simulink model "W01_Base_Map_cs"  (R2019a)
settings: Solver=FixedStepDiscrete  StartTime=0.0  StopTime=inf  FixedStep=1/20  RelTol=1e-3
PreLoadFcn:
  | mbxruntime.callbacks.PreLoadFcn(bdroot);
  | check_NUTS_defined
  | model_closed = 0;
  | assignin('base',['model_closed_' bdroot],false);
PostLoadFcn:
  | mbxruntime.callbacks.PostLoadFcn(bdroot);
InitFcn:
  | mbxruntime.callbacks.InitFcn(bdroot);
StartFcn:
  | mbxruntime.callbacks.StartFcn(bdroot);
StopFcn:
  | mbxruntime.callbacks.StopFcn(bdroot);;
  | 
model workspace: external: MAT-File (data not in the file)
undefined symbols (not defined in the file or in its folder): actors_poses, adeye_msgs, categorized_poses, DiscIntNeverNeededParam, geometry_msgs, Header, InitImageOutputDir, mbxruntime, pose_otherCar, PoseArray, Poses, Poses_SL_Info, tabledata, W01_Base_Map_cs_004987d4dd39f9b6, W01_Base_Map_cs_00cc66853e964a64, W01_Base_Map_cs_00f75b713170549a, W01_Base_Map_cs_01472650a6655f66, W01_Base_Map_cs_021eada97d6d5412, W01_Base_Map_cs_0288936122941f67, W01_Base_Map_cs_03728bc5c0f611d1, W01_Base_Map_cs_03729b7883682eca, W01_Base_Map_cs_03935175e827b825, W01_Base_Map_cs_03ecb5a7ceaf36f1, W01_Base_Map_cs_04544dd62153117c, W01_Base_Map_cs_04f0838a8dce3a91, W01_Base_Map_cs_05c6883b663017e6, W01_Base_Map_cs_074ff6b44c8e4b42, W01_Base_Map_cs_0850adb5f9b52847, W01_Base_Map_cs_09b4416d284a38c0, W01_Base_Map_cs_09f1a8cccf5dc476, W01_Base_Map_cs_0a863e6a78242047, W01_Base_Map_cs_0b51b2edfb6b21eb, W01_Base_Map_cs_0c25b2d8edd3fbea, W01_Base_Map_cs_0cec291d859792a3, W01_Base_Map_cs_0d48999ceb9def0a, W01_Base_Map_cs_1054e386bc2b89f8, W01_Base_Map_cs_129d7fd29679c9e4, W01_Base_Map_cs_1557dafebe6eb5e3, W01_Base_Map_cs_155bf6da17508b9f, W01_Base_Map_cs_1619aae3285d69a6, W01_Base_Map_cs_18faf784f59d6ded, W01_Base_Map_cs_190ae931cd3b3df1, W01_Base_Map_cs_1a47612a95ab18a1, W01_Base_Map_cs_1a96581334d27a16, W01_Base_Map_cs_1b9c28e1ad91b987, W01_Base_Map_cs_1bd80946b29cc249, W01_Base_Map_cs_1bf8c5472ecd97cc, W01_Base_Map_cs_1c047b8f6e9a46e9, W01_Base_Map_cs_1c4e91c4c8848966, W01_Base_Map_cs_1dfe629d3c3a34d6, W01_Base_Map_cs_1e00e80d4fa95f87, W01_Base_Map_cs_1e67a7d0e7e33a10, W01_Base_Map_cs_1e994bb86296e53e, W01_Base_Map_cs_1f3d28b65a209a81, W01_Base_Map_cs_1f4ddfcaed2bdfa2, W01_Base_Map_cs_20e6a062a8bf989a, W01_Base_Map_cs_210ba2feda70a68e, W01_Base_Map_cs_211f71a4af886b52, W01_Base_Map_cs_2177d1459a678375, W01_Base_Map_cs_21a90c8036f5a434 ... (+289)
libraries: PreScanSimulinkLibrary x112, robotcorelib x55, adeye_lib x46, simulink x31, simulink_extras x24, robotlib x3, PreScanUsefulBlocks x1
(part 1 of 32)
CloseFcn:
  | mbxruntime.callbacks.CloseFcn(bdroot);
  | evalin('base',['clear model_closed_' bdroot]);
  | model_closed = 1;
settings Model: Creator=PRESCAN  LastModifiedBy=adeye
settings DataIOCC: LimitDataPoints=on  SaveFormat=Array  SignalLoggingSaveFormat=ModelDataLogs  ReturnWorkspaceOutputs=off
settings OptimizationCC: DefaultParameterBehavior=Inlined  ExpressionDepthLimit=2147483647  InitFltsAndDblsToZero=on  LifeSpan=inf
settings DebuggingCC: SaveWithParameterizedLinksMsg=none  UnderspecifiedInitializationDetection=Classic  MergeDetectMultiDrivingBlocksExec=none  SignalResolutionControl=TryResolveAllWithWarning  MultiTaskDSMMsg=warning  MultiTaskCondExecSysMsg=none  FcnCallInpInsideContextMsg=warning  StateNameClashWarn=warning  SFUnexpectedBacktrackingDiag=warning  SFNoUnconditionalDefaultTransitionDiag=warning  SFExecutionAtInitializationDiag=none  ArithmeticOperatorsInVariantConditions=warning
settings HardwareCC: ProdBitPerPointer=32  ProdBitPerSizeT=32  ProdBitPerPtrDiffT=32  ProdLargestAtomicFloat=None  ProdIntDivRoundTo=Undefined  ProdEndianess=Unspecified  ProdWordSize=32  ProdHWDeviceType=32-bit Generic
settings ModelReferenceCC: UpdateModelReferenceTargets=IfOutOfDate  PropagateSignalLabelsOutOfModel=off
settings SFSimCC: SimUseLocalCustomCode=off  SimParseCustomCode=off
settings SFSimCC: SimCustomHeaderCode=|
  | #include "prescan.h"
  | #include "prescan_platform.h"
  | #include "prescan_aimsunturnindicatorsetter_data.h"
settings RTWCC: RTWUseLocalCustomCode=off
settings CodeAppCC: StateflowObjectComments=on
settings GRTTargetCC: TargetFcnLib=ansi_tfl_tmw.mat  TargetLangStandard=C89/C90 (ANSI)  GeneratePreprocessorConditionals=Disable all  CombineOutputUpdateFcns=off  GRTInterface=on
settings ConfigComp: CovMetricSettings=dw  CovHtmlReporting=on  CovSaveCumulativeToWorkspaceVar=on  CovSaveSingleToWorkspaceVar=on  CovExternalEMLEnable=off  CovSFcnEnable=off

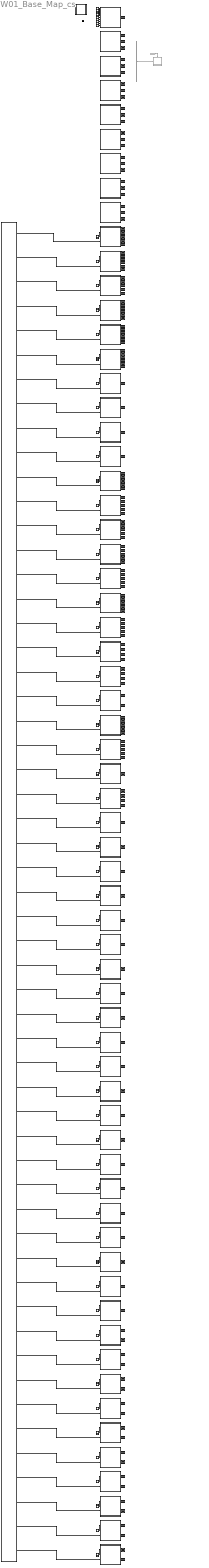
== system W01_Base_Map_cs ==
  note: Regenerate
  note: Simulink Mode
  note: Open Useful Blocks
  note: 2020.4.0
  note: Version:
  note: Author(s):
  note: Adeye
  note: Descriptive text:
  note: N.A.
  note: Demo Help
  note: ====== Num ID ====== 91 93 94 95 96 97 76 77 78 79 80 82 83 81 37 109 115 116 117 118 119 120 121 122 123 124 125 126 127 128 ====== Num ID ====== 129 130 131 132 133 134 135 136 137 138 139 140 141 142 143 144 145 146 147 148 149 150 151 152 153 154 155 156 157 110 ====== Num ID ====== 159 160 161 162 163 164 165 166 167
  note: ============= OBU-Beacon ID ============= ============= OBU-Beacon ID ============= ============= OBU-Beacon ID =============
  note: ======= Type ID ======= 12 12 12 12 12 12 15 15 15 15 15 15 15 15 4 4 4 4 4 4 2 2 1 1 4 4 4 4 4 4 ======= Type ID ======= 4 4 4 4 4 4 4 4 1 1 1 1 1 1 1 1 1 1 1 1 1 1 1 1 1 1 2 2 2 4 ======= Type ID ======= 4 4 4 4 4 4 4 4 4
  note: ================ Type Tag ================ Building Building Building Building Building Building Animated traffic sign Animated traffic sign Animated traffic sign Animated traffic sign Animated traffic sign Animated traffic sign Animated traffic sign Animated traffic sign Human Human Human Human Human Human Motor Motor Car Car Human Human Human Human Human Human ================ Type Tag ================ Human Human Human Human Human Human Human Human Car Car Car Car Car Car Car Car Car Car Car Car Car Car Car Car Car Car Motor Motor Motor Human ================ Type Tag ================ Human Human Human Human Human Human Human Human Human
  note: == SD == Y Y Y Y Y Y Y Y Y Y Y Y Y Y Y Y Y Y Y Y Y Y Y Y Y Y Y Y Y Y == SD == Y Y Y Y Y Y Y Y Y Y Y Y Y Y Y Y Y Y Y Y Y Y Y Y Y Y Y Y Y Y == SD == Y Y Y Y Y Y Y Y Y
  note: == CD == N N N N N N N N N N N N N N N N N N N N N N N N N N N N N N == CD == N N N N N N N N N N N N N N N N N N N N N N N N N N N N N N == CD == N N N N N N N N N
  note: ================================== Name ================================== HouseOld3_1 HouseOld4_1 HouseOld5_1 School_1 OfficeBrownFlat_1 OfficeBrownTall2_1 TrafficLightRoadSideNL_1 TrafficLightRoadSideNL_2 TrafficLightRoadSideNL_3 TrafficLightRoadSideNL_4 TrafficLightRoadSideNL_5 TrafficLightRoadSideNL_7 TrafficLightRoadSideNL_8 TrafficLightRoadSideNL_6 Female_Regular_1 Male_wLargeBackpack_1 Male_wBackpack_1 Male_ShoppingBag_1 Male_LargeShoulderSuitcase_1 Male_wLongCoat_1 Honda_Pan_European_Motorcycle_With_Driver_1 Sports_Bike_wDriver_1 Tesla_Model_3_1 Volvo_XC60_1 Boy_150_1 Child_Overweight_1 Female_Overweight_1 Female_wBuggy_1 Female_wLongCoat_1 Female_wRaincoat_1 ================================== Name ================================== Male_African_1 Male_Old_White_WithStick_1 Male_Overweight_1 Male_wSuit_1 Male_200_1 Man_250_1 Male_Old_White_WithWalker_1 Male_Old_White_WithWalkerWithWheels_1 Audi_A3_1 Audi_A8_Sedan_2 BMW_Z3_Convertible_1 Citroen_C3_Hatchback_2 Fiat_Bravo_Hatchback_1 Ford_Fiesta_Hatchback_2 Ford_Focus_Stationwagon_1 Lexus_GS_450h_F_Sport_Sedan_1 Lexus_LS_600h_F_Sport_1 Mazda_RX8_Coupe_1 Roewe_550_S_Sedan_1 Toyota_Previa_MPV_1 Toyota_Prius_Sedan_1 Toyota_Yaris_Hatchback_1 Wuling_Hongguang_1 Toyota_Yaris_Hatchback_2 Citroen_C3_Hatchback_3 Audi_A3_2 Sports_Bike_wDriver_2 Sports_Bike_wDriver_3 Honda_Pan_European_Motorcycle_With_Driver_2 Male_CyclingCyclist_1 ================================== Name ================================== Male_CyclingCyclist_2 Male_CyclingCyclist_3 Male_CyclingCyclist_4 Male_CyclingCyclist_5 Male_CyclingCyclist_6 Male_CyclingCyclist_7 Male_CyclingCyclist_8 Male_CyclingCyclist_9 Male_CyclingCyclist_10
  ANIM_Boy_150_1 : Subsystem  Tag=actuator/AnimationOutport  Priority=0  LoadFcn=load('PreScanAnimActuatorData.mat')  mask(PreScan Sink Block: State Animation){}
      mask help: The Human Animation port allows the human to walk, run or bend
      settings: OpenFcn=open_system([gcb '/Actuator'],'mask')
      mask Help: eval('openHelp(239)')
      mask Display: image(imread('HumanAnimated.jpg'))
  ANIM_Child_Overweight_1 : Subsystem  Tag=actuator/AnimationOutport  Priority=0  LoadFcn=load('PreScanAnimActuatorData.mat')  mask(PreScan Sink Block: State Animation){}
      mask help: The Human Animation port allows the human to walk, run or bend
      settings: OpenFcn=open_system([gcb '/Actuator'],'mask')
      mask Help: eval('openHelp(239)')
      mask Display: image(imread('HumanAnimated.jpg'))
  ANIM_Female_Overweight_1 : Subsystem  Tag=actuator/AnimationOutport  Priority=0  LoadFcn=load('PreScanAnimActuatorData.mat')  mask(PreScan Sink Block: State Animation){}
      mask help: The Human Animation port allows the human to walk, run or bend
      settings: OpenFcn=open_system([gcb '/Actuator'],'mask')
      mask Help: eval('openHelp(239)')
      mask Display: image(imread('HumanAnimated.jpg'))
  ANIM_Female_Regular_1 : Subsystem  Tag=actuator/AnimationOutport  Priority=0  LoadFcn=load('PreScanAnimActuatorData.mat')  mask(PreScan Sink Block: State Animation){}
      mask help: The Human Animation port allows the human to walk, run or bend
      settings: OpenFcn=open_system([gcb '/Actuator'],'mask')
      mask Help: eval('openHelp(239)')
      mask Display: image(imread('HumanAnimated.jpg'))
  ANIM_Female_wBuggy_1 : Subsystem  Tag=actuator/AnimationOutport  Priority=0  LoadFcn=load('PreScanAnimActuatorData.mat')  mask(PreScan Sink Block: State Animation){}
      mask help: The Human Animation port allows the human to walk, run or bend
      settings: OpenFcn=open_system([gcb '/Actuator'],'mask')
      mask Help: eval('openHelp(239)')
      mask Display: image(imread('HumanAnimated.jpg'))
  ANIM_Female_wLongCoat_1 : Subsystem  Tag=actuator/AnimationOutport  Priority=0  LoadFcn=load('PreScanAnimActuatorData.mat')  mask(PreScan Sink Block: State Animation){}
      mask help: The Human Animation port allows the human to walk, run or bend
      settings: OpenFcn=open_system([gcb '/Actuator'],'mask')
      mask Help: eval('openHelp(239)')
      mask Display: image(imread('HumanAnimated.jpg'))
  ANIM_Female_wRaincoat_1 : Subsystem  Tag=actuator/AnimationOutport  Priority=0  LoadFcn=load('PreScanAnimActuatorData.mat')  mask(PreScan Sink Block: State Animation){}
      mask help: The Human Animation port allows the human to walk, run or bend
      settings: OpenFcn=open_system([gcb '/Actuator'],'mask')
      mask Help: eval('openHelp(239)')
      mask Display: image(imread('HumanAnimated.jpg'))
  ANIM_Male_200_1 : Subsystem  Tag=actuator/AnimationOutport  Priority=0  LoadFcn=load('PreScanAnimActuatorData.mat')  mask(PreScan Sink Block: State Animation){}
      mask help: The Human Animation port allows the human to walk, run or bend
      settings: OpenFcn=open_system([gcb '/Actuator'],'mask')
      mask Help: eval('openHelp(239)')
      mask Display: image(imread('HumanAnimated.jpg'))
  ANIM_Male_African_1 : Subsystem  Tag=actuator/AnimationOutport  Priority=0  LoadFcn=load('PreScanAnimActuatorData.mat')  mask(PreScan Sink Block: State Animation){}
      mask help: The Human Animation port allows the human to walk, run or bend
      settings: OpenFcn=open_system([gcb '/Actuator'],'mask')
      mask Help: eval('openHelp(239)')
      mask Display: image(imread('HumanAnimated.jpg'))
  ANIM_Male_CyclingCyclist_1 : Subsystem  Tag=actuator/AnimationOutport  Priority=0  LoadFcn=load('PreScanAnimActuatorData.mat')  mask(PreScan Sink Block: State Animation){}
      mask help: The Human Animation port allows the human to walk, run or bend
      settings: OpenFcn=open_system([gcb '/Actuator'],'mask')
      mask Help: eval('openHelp(239)')
      mask Display: image(imread('HumanAnimated.jpg'))
  ANIM_Male_CyclingCyclist_10 : Subsystem  Tag=actuator/AnimationOutport  Priority=0  LoadFcn=load('PreScanAnimActuatorData.mat')  mask(PreScan Sink Block: State Animation){}
      mask help: The Human Animation port allows the human to walk, run or bend
      settings: OpenFcn=open_system([gcb '/Actuator'],'mask')
      mask Help: eval('openHelp(239)')
      mask Display: image(imread('HumanAnimated.jpg'))
  ANIM_Male_CyclingCyclist_2 : Subsystem  Tag=actuator/AnimationOutport  Priority=0  LoadFcn=load('PreScanAnimActuatorData.mat')  mask(PreScan Sink Block: State Animation){}
      mask help: The Human Animation port allows the human to walk, run or bend
      settings: OpenFcn=open_system([gcb '/Actuator'],'mask')
      mask Help: eval('openHelp(239)')
      mask Display: image(imread('HumanAnimated.jpg'))
  ANIM_Male_CyclingCyclist_3 : Subsystem  Tag=actuator/AnimationOutport  Priority=0  LoadFcn=load('PreScanAnimActuatorData.mat')  mask(PreScan Sink Block: State Animation){}
      mask help: The Human Animation port allows the human to walk, run or bend
      settings: OpenFcn=open_system([gcb '/Actuator'],'mask')
      mask Help: eval('openHelp(239)')
      mask Display: image(imread('HumanAnimated.jpg'))
  ANIM_Male_CyclingCyclist_4 : Subsystem  Tag=actuator/AnimationOutport  Priority=0  LoadFcn=load('PreScanAnimActuatorData.mat')  mask(PreScan Sink Block: State Animation){}
      mask help: The Human Animation port allows the human to walk, run or bend
      settings: OpenFcn=open_system([gcb '/Actuator'],'mask')
      mask Help: eval('openHelp(239)')
      mask Display: image(imread('HumanAnimated.jpg'))
  ANIM_Male_CyclingCyclist_5 : Subsystem  Tag=actuator/AnimationOutport  Priority=0  LoadFcn=load('PreScanAnimActuatorData.mat')  mask(PreScan Sink Block: State Animation){}
      mask help: The Human Animation port allows the human to walk, run or bend
      settings: OpenFcn=open_system([gcb '/Actuator'],'mask')
      mask Help: eval('openHelp(239)')
      mask Display: image(imread('HumanAnimated.jpg'))
  ANIM_Male_CyclingCyclist_6 : Subsystem  Tag=actuator/AnimationOutport  Priority=0  LoadFcn=load('PreScanAnimActuatorData.mat')  mask(PreScan Sink Block: State Animation){}
      mask help: The Human Animation port allows the human to walk, run or bend
      settings: OpenFcn=open_system([gcb '/Actuator'],'mask')
      mask Help: eval('openHelp(239)')
      mask Display: image(imread('HumanAnimated.jpg'))
  ANIM_Male_CyclingCyclist_7 : Subsystem  Tag=actuator/AnimationOutport  Priority=0  LoadFcn=load('PreScanAnimActuatorData.mat')  mask(PreScan Sink Block: State Animation){}
      mask help: The Human Animation port allows the human to walk, run or bend
      settings: OpenFcn=open_system([gcb '/Actuator'],'mask')
      mask Help: eval('openHelp(239)')
      mask Display: image(imread('HumanAnimated.jpg'))
  ANIM_Male_CyclingCyclist_8 : Subsystem  Tag=actuator/AnimationOutport  Priority=0  LoadFcn=load('PreScanAnimActuatorData.mat')  mask(PreScan Sink Block: State Animation){}
      mask help: The Human Animation port allows the human to walk, run or bend
      settings: OpenFcn=open_system([gcb '/Actuator'],'mask')
      mask Help: eval('openHelp(239)')
      mask Display: image(imread('HumanAnimated.jpg'))
  ANIM_Male_CyclingCyclist_9 : Subsystem  Tag=actuator/AnimationOutport  Priority=0  LoadFcn=load('PreScanAnimActuatorData.mat')  mask(PreScan Sink Block: State Animation){}
      mask help: The Human Animation port allows the human to walk, run or bend
      settings: OpenFcn=open_system([gcb '/Actuator'],'mask')
      mask Help: eval('openHelp(239)')
      mask Display: image(imread('HumanAnimated.jpg'))
  ANIM_Male_LargeShoulderSuitcase_1 : Subsystem  Tag=actuator/AnimationOutport  Priority=0  LoadFcn=load('PreScanAnimActuatorData.mat')  mask(PreScan Sink Block: State Animation){}
      mask help: The Human Animation port allows the human to walk, run or bend
      settings: OpenFcn=open_system([gcb '/Actuator'],'mask')
      mask Help: eval('openHelp(239)')
      mask Display: image(imread('HumanAnimated.jpg'))
  ANIM_Male_Overweight_1 : Subsystem  Tag=actuator/AnimationOutport  Priority=0  LoadFcn=load('PreScanAnimActuatorData.mat')  mask(PreScan Sink Block: State Animation){}
      mask help: The Human Animation port allows the human to walk, run or bend
      settings: OpenFcn=open_system([gcb '/Actuator'],'mask')
      mask Help: eval('openHelp(239)')
      mask Display: image(imread('HumanAnimated.jpg'))
  ANIM_Male_ShoppingBag_1 : Subsystem  Tag=actuator/AnimationOutport  Priority=0  LoadFcn=load('PreScanAnimActuatorData.mat')  mask(PreScan Sink Block: State Animation){}
      mask help: The Human Animation port allows the human to walk, run or bend
      settings: OpenFcn=open_system([gcb '/Actuator'],'mask')
      mask Help: eval('openHelp(239)')
      mask Display: image(imread('HumanAnimated.jpg'))
  ANIM_Male_wBackpack_1 : Subsystem  Tag=actuator/AnimationOutport  Priority=0  LoadFcn=load('PreScanAnimActuatorData.mat')  mask(PreScan Sink Block: State Animation){}
      mask help: The Human Animation port allows the human to walk, run or bend
      settings: OpenFcn=open_system([gcb '/Actuator'],'mask')
      mask Help: eval('openHelp(239)')
      mask Display: image(imread('HumanAnimated.jpg'))
  ANIM_Male_wLargeBackpack_1 : Subsystem  Tag=actuator/AnimationOutport  Priority=0  LoadFcn=load('PreScanAnimActuatorData.mat')  mask(PreScan Sink Block: State Animation){}
      mask help: The Human Animation port allows the human to walk, run or bend
      settings: OpenFcn=open_system([gcb '/Actuator'],'mask')
      mask Help: eval('openHelp(239)')
      mask Display: image(imread('HumanAnimated.jpg'))
  ANIM_Male_wLongCoat_1 : Subsystem  Tag=actuator/AnimationOutport  Priority=0  LoadFcn=load('PreScanAnimActuatorData.mat')  mask(PreScan Sink Block: State Animation){}
      mask help: The Human Animation port allows the human to walk, run or bend
      settings: OpenFcn=open_system([gcb '/Actuator'],'mask')
      mask Help: eval('openHelp(239)')
      mask Display: image(imread('HumanAnimated.jpg'))
  ANIM_Male_wSuit_1 : Subsystem  Tag=actuator/AnimationOutport  Priority=0  LoadFcn=load('PreScanAnimActuatorData.mat')  mask(PreScan Sink Block: State Animation){}
      mask help: The Human Animation port allows the human to walk, run or bend
      settings: OpenFcn=open_system([gcb '/Actuator'],'mask')
      mask Help: eval('openHelp(239)')
      mask Display: image(imread('HumanAnimated.jpg'))
  ANIM_Man_250_1 : Subsystem  Tag=actuator/AnimationOutport  Priority=0  LoadFcn=load('PreScanAnimActuatorData.mat')  mask(PreScan Sink Block: State Animation){}
      mask help: The Human Animation port allows the human to walk, run or bend
      settings: OpenFcn=open_system([gcb '/Actuator'],'mask')
      mask Help: eval('openHelp(239)')
      mask Display: image(imread('HumanAnimated.jpg'))
  Audi_A3_1 : Subsystem  Tag=WorldObjectSubSystem  InitFcn=UniqueId = '29061';
      mask init:
      | modelPath = GenericModelHelper.getGenericModelFilePath('ModelDepo','Vehicles\Audi_A3\Audi_A3.pgmb','e624684529bbc602b96708a92995a42d');imagePath = GenericModelHelper.getCompilationPicture(modelPath, 'Audi_A3.png');
      mask Display: image(imread(imagePath));color('white');text(0, 0, ' ID=137\n')
  Audi_A3_2 : Subsystem  Tag=WorldObjectSubSystem  InitFcn=UniqueId = '29078';
      mask init: same as W01_Base_Map_cs/Audi_A3_1
      mask Display: image(imread(imagePath));color('white');text(0, 0, ' ID=154\n')
  Audi_A8_Sedan_2 : Subsystem  Tag=WorldObjectSubSystem  InitFcn=UniqueId = '29062';
      mask init:
      | modelPath = GenericModelHelper.getGenericModelFilePath('ModelDepo','Vehicles\Audi_A8\Audi_A8.pgmb','e33fe1ddcf3e8ae97caccbc8f2fa74ac');imagePath = GenericModelHelper.getCompilationPicture(modelPath, 'Audi_A8_HighPoly.png');
      mask Display: image(imread(imagePath));color('white');text(0, 0, ' ID=138\n')
  BMW_X5_SUV_1 : Subsystem  Tag=WorldObjectSubSystem  InitFcn=UniqueId = '9040';
      mask init:
      | modelPath = GenericModelHelper.getGenericModelFilePath('ModelDepo','Vehicles\BMW_X5\BMW_X5.pgmb','bfeb1c11467705ab888b3011684c848b');imagePath = GenericModelHelper.getCompilationPicture(modelPath, 'BMW_X5_HighPoly.png');
      mask Display: image(imread(imagePath));color('white');text(0, 0, ' ID=55\n')
  BMW_Z3_Convertible_1 : Subsystem  Tag=WorldObjectSubSystem  InitFcn=UniqueId = '29063';
      mask init:
      | modelPath = GenericModelHelper.getGenericModelFilePath('ModelDepo','Vehicles\BMW_Z3\BMW_Z3.pgmb','9e6af5cc2d86218dad43975fd3a29d11');imagePath = GenericModelHelper.getCompilationPicture(modelPath, 'BMW_Z3_HighPoly.png');
      mask Display: image(imread(imagePath));color('white');text(0, 0, ' ID=139\n')
  Boy_150_1 : Subsystem  Tag=WorldObjectSubSystem  InitFcn=UniqueId = '29047';
      mask init:
      | modelPath = GenericModelHelper.getGenericModelFilePath('ModelDepo','Humans\Boy_150\Boy_150.pgmb','fbfe73b6a39381f55b0a93538b37a6f8');imagePath = GenericModelHelper.getCompilationPicture(modelPath, 'Boy_150.png');
      mask Display: image(imread(imagePath));color('white');text(0, 0, ' ID=123\n')
  Camera_1 : Subsystem  Tag=sensor/Camera/CameraSensor  Priority=30  mask(PreScan Source Block: Camera Sensor){}
      mask help: The Camera Sensor provides a color or monochrome image.
      settings: OpenFcn=open_system([gcb '/Sensor'],'mask')
      mask Help: eval('openHelp(457)')
      mask Display: image(imread('CameraSensor.png'))
  Camera_2 : Subsystem  Tag=sensor/Camera/CameraSensor  Priority=30  mask(PreScan Source Block: Camera Sensor){}
      mask help: The Camera Sensor provides a color or monochrome image.
      settings: OpenFcn=open_system([gcb '/Sensor'],'mask')
      mask Help: eval('openHelp(457)')
      mask Display: image(imread('CameraSensor.png'))
  Camera_tl : Subsystem  Tag=sensor/Camera/CameraSensor  Priority=30  mask(PreScan Source Block: Camera Sensor){}
      mask help: The Camera Sensor provides a color or monochrome image.
      settings: OpenFcn=open_system([gcb '/Sensor'],'mask')
      mask Help: eval('openHelp(457)')
      mask Display: image(imread('CameraSensor.png'))
  Child_Overweight_1 : Subsystem  Tag=WorldObjectSubSystem  InitFcn=UniqueId = '29048';
      mask init:
      | modelPath = GenericModelHelper.getGenericModelFilePath('ModelDepo','Humans\ChildOverweight\Child_Overweight.pgmb','8bbd7c9b287bc99b5fac267955a0e349');imagePath = GenericModelHelper.getCompilationPicture(modelPath, 'ChildOverweight.png');
      mask Display: image(imread(imagePath));color('white');text(0, 0, ' ID=124\n')
  Citroen_C3_Hatchback_2 : Subsystem  Tag=WorldObjectSubSystem  InitFcn=UniqueId = '29064';
      mask init:
      | modelPath = GenericModelHelper.getGenericModelFilePath('ModelDepo','Vehicles\Citroen_C3\Citroen_C3.pgmb','e804ced06d50dbfc6a2202ab3ad01b0c');imagePath = GenericModelHelper.getCompilationPicture(modelPath, 'Citroen_C3_HighPoly.png');
      mask Display: image(imread(imagePath));color('white');text(0, 0, ' ID=140\n')
  Citroen_C3_Hatchback_3 : Subsystem  Tag=WorldObjectSubSystem  InitFcn=UniqueId = '29077';
      mask init: same as W01_Base_Map_cs/Citroen_C3_Hatchback_2
      mask Display: image(imread(imagePath));color('white');text(0, 0, ' ID=153\n')
  Controller : Subsystem  Description=8A3CD2955739A82C886C20AE3E253D78460D53180EE2C1B14CC08DF75A70BE77  Priority=-1  LoadFcn=load PreScanControllerData  mask(PreScan Simulation Controller){prescanversion='2020.4.0', ModelReferencing=off, TimeStep=1/20, ControlMode=0, PreScanExecutionMode=on, ControllerCount=0, ControllerIndex=0, ControllerOptions=''}
      mask prompts: prescanversion "PreScan Version"; ModelReferencing "Use Model Referencing"; TimeStep "Upload Period [s]"; ControlMode "Control Mode"; PreScanExecutionMode "Execution Mode"; ControllerCount "Controller Count"; ControllerIndex "Controller Index"; ControllerOptions "Controller Options"
      mask help: Please do not remove this block from the compilation sheet, as it connects the model to the PreScan environment.
      mask init:
      | model = bdroot(gcb);
      | ExperimentFile = mbxruntime.findExperimentFile(model,true); %relative path
      | 
      | [d1, d2, d3, prescandata] = prescan_Settings();
      | ModelDepo = fullfile(prescandata,'ModelDepo'); 
      | 
      | RTmode = mbxruntime.getRTMode(model);
      | 
      | SimulationMode = get_param(bdroot,'SimulationMode');
      | if strcmp(SimulationMode, 'rapid-accelerator')
      |     SimulationMode = 'external';
      | end
      | TargetName = get_param(bdroot,'SystemTargetFile');
      settings: ModelCloseFcn=assignin('base',['model_closed_' bdroot],true);
      mask Help: eval('openHelp(812)')
      mask Display: image(imread('prescanlogo.ico'))
  Female_Overweight_1 : Subsystem  Tag=WorldObjectSubSystem  InitFcn=UniqueId = '29049';
      mask init:
      | modelPath = GenericModelHelper.getGenericModelFilePath('ModelDepo','Humans\FemaleOverweight\Female_Overweight.pgmb','3364bded42c189aacfb51fba9ba11ae6');imagePath = GenericModelHelper.getCompilationPicture(modelPath, 'FemaleOverweight.png');
      mask Display: image(imread(imagePath));color('white');text(0, 0, ' ID=125\n')
  Female_Regular_1 : Subsystem  Tag=WorldObjectSubSystem  InitFcn=UniqueId = '28384';
      mask init:
      | modelPath = GenericModelHelper.getGenericModelFilePath('ModelDepo','Humans\FemaleRegular\Female_Regular.pgmb','a60942a07dc01011c3a5e5a36c910370');imagePath = GenericModelHelper.getCompilationPicture(modelPath, 'FemaleRegular.png');
      mask Display: image(imread(imagePath));color('white');text(0, 0, ' ID=37\n')
  Female_wBuggy_1 : Subsystem  Tag=WorldObjectSubSystem  InitFcn=UniqueId = '29050';
      mask init:
      | modelPath = GenericModelHelper.getGenericModelFilePath('ModelDepo','Humans\FemaleBuggy\Female_wBuggy.pgmb','496cbc283fa2ef39016d6050ab389860');imagePath = GenericModelHelper.getCompilationPicture(modelPath, 'FemaleBuggy.png');
      mask Display: image(imread(imagePath));color('white');text(0, 0, ' ID=126\n')
  Female_wLongCoat_1 : Subsystem  Tag=WorldObjectSubSystem  InitFcn=UniqueId = '29051';
      mask init:
      | modelPath = GenericModelHelper.getGenericModelFilePath('ModelDepo','Humans\Female_wLongCoat\Female_wLongCoat.pgmb','055d8c3918aa618f0232f0160254dd2c');imagePath = GenericModelHelper.getCompilationPicture(modelPath, 'Female_wLongCoat.png');
      mask Display: image(imread(imagePath));color('white');text(0, 0, ' ID=127\n')
  Female_wRaincoat_1 : Subsystem  Tag=WorldObjectSubSystem  InitFcn=UniqueId = '29052';
      mask init:
      | modelPath = GenericModelHelper.getGenericModelFilePath('ModelDepo','Humans\FemaleRaincoat\Female_wRaincoat.pgmb','6cfcbcafb642f393cffaa2cc5bebeb23');imagePath = GenericModelHelper.getCompilationPicture(modelPath, 'FemaleRaincoat.png');
      mask Display: image(imread(imagePath));color('white');text(0, 0, ' ID=128\n')
  Fiat_Bravo_Hatchback_1 : Subsystem  Tag=WorldObjectSubSystem  InitFcn=UniqueId = '29065';
      mask init:
      | modelPath = GenericModelHelper.getGenericModelFilePath('ModelDepo','Vehicles\Fiat_Bravo\Fiat_Bravo.pgmb','a97eb0ec4093646e5d079d2ab9a2eab7');imagePath = GenericModelHelper.getCompilationPicture(modelPath, 'Fiat_Bravo_HighPoly.png');
      mask Display: image(imread(imagePath));color('white');text(0, 0, ' ID=141\n')
  Ford_Fiesta_Hatchback_2 : Subsystem  Tag=WorldObjectSubSystem  InitFcn=UniqueId = '29066';
      mask init:
      | modelPath = GenericModelHelper.getGenericModelFilePath('ModelDepo','Vehicles\Ford_Fiesta\Ford_Fiesta.pgmb','fe2c7a73e0a60cba76689b71cd1bb76a');imagePath = GenericModelHelper.getCompilationPicture(modelPath, 'Ford_Fiesta_HighPoly.png');
      mask Display: image(imread(imagePath));color('white');text(0, 0, ' ID=142\n')
  Ford_Focus_Stationwagon_1 : Subsystem  Tag=WorldObjectSubSystem  InitFcn=UniqueId = '29067';
      mask init:
      | modelPath = GenericModelHelper.getGenericModelFilePath('ModelDepo','Vehicles\Ford_Focus_Wagon\Ford_Focus_Wagon.pgmb','daf8bd73c88a9bb5f3f179d705958474');imagePath = GenericModelHelper.getCompilationPicture(modelPath, 'Ford_Focus_Wagon.png');
      mask Display: image(imread(imagePath));color('white');text(0, 0, ' ID=143\n')
  From9 : From  Commented=on  GotoTag=other
  Honda_Pan_European_Motorcycle_With_Driver_1 : Subsystem  Tag=WorldObjectSubSystem  InitFcn=UniqueId = '29035';
      mask init:
      | modelPath = GenericModelHelper.getGenericModelFilePath('ModelDepo','Vehicles\Honda_Pan_European_With_Driver\Honda_Pan_European_With_Driver.pgmb','87ba31455683eb3e7a0d63db23b59554');imagePath = GenericModelHelper.getCompilationPicture(modelPath, 'Honda_Pan_European_HighPoly_With_Driver.png');
      mask Display: image(imread(imagePath));color('white');text(0, 0, ' ID=119\n')
  Honda_Pan_European_Motorcycle_With_Driver_2 : Subsystem  Tag=WorldObjectSubSystem  InitFcn=UniqueId = '29108';
      mask init: same as W01_Base_Map_cs/Honda_Pan_European_Motorcycle_With_Driver_1
      mask Display: image(imread(imagePath));color('white');text(0, 0, ' ID=157\n')
  Lexus_GS_450h_F_Sport_Sedan_1 : Subsystem  Tag=WorldObjectSubSystem  InitFcn=UniqueId = '29068';
      mask init:
      | modelPath = GenericModelHelper.getGenericModelFilePath('ModelDepo','Vehicles\Lexus_GS_450h_F_Sport\Lexus_GS_450h_F_Sport.pgmb','fb0997f68165d6ffd45e3f9a26a4fc2e');imagePath = GenericModelHelper.getCompilationPicture(modelPath, 'Lexus_GS_450h_F_Sport_HighPoly.png');
      mask Display: image(imread(imagePath));color('white');text(0, 0, ' ID=144\n')
  Lexus_LS_600h_F_Sport_1 : Subsystem  Tag=WorldObjectSubSystem  InitFcn=UniqueId = '29069';
      mask init:
      | modelPath = GenericModelHelper.getGenericModelFilePath('ModelDepo','Vehicles\Lexus_LS_600h_F_Sport\Lexus_LS_600h_F_Sport.pgmb','27e45258e125e5b1a8b40c825c13d9fe');imagePath = GenericModelHelper.getCompilationPicture(modelPath, 'Lexus_LS_600h_F_Sport_HighPoly.png');
      mask Display: image(imread(imagePath));color('white');text(0, 0, ' ID=145\n')
  Male_200_1 : Subsystem  Tag=WorldObjectSubSystem  InitFcn=UniqueId = '29057';
      mask init:
      | modelPath = GenericModelHelper.getGenericModelFilePath('ModelDepo','Humans\Male200\Male_200.pgmb','97a2394f555eb1924c7e25baff3f8b80');imagePath = GenericModelHelper.getCompilationPicture(modelPath, 'Male200.png');
      mask Display: image(imread(imagePath));color('white');text(0, 0, ' ID=133\n')
  Male_African_1 : Subsystem  Tag=WorldObjectSubSystem  InitFcn=UniqueId = '29053';
      mask init:
      | modelPath = GenericModelHelper.getGenericModelFilePath('ModelDepo','Humans\MaleAfrican\Male_African.pgmb','b904c575fa50030e0f2032b1e76d9d83');imagePath = GenericModelHelper.getCompilationPicture(modelPath, 'MaleAfrican.png');
      mask Display: image(imread(imagePath));color('white');text(0, 0, ' ID=129\n')
  Male_CyclingCyclist_1 : Subsystem  Tag=WorldObjectSubSystem  InitFcn=UniqueId = '29109';
      mask init:
      | modelPath = GenericModelHelper.getGenericModelFilePath('ModelDepo','Humans\MaleCyclingCyclist\Male_CyclingCyclist.pgmb','4da2b938887cc3bba922388c76512291');imagePath = GenericModelHelper.getCompilationPicture(modelPath, 'MaleCyclingCyclist.png');
      mask Display: image(imread(imagePath));color('white');text(0, 0, ' ID=110\n')
  Male_CyclingCyclist_10 : Subsystem  Tag=WorldObjectSubSystem  InitFcn=UniqueId = '29119';
      mask init: same as W01_Base_Map_cs/Male_CyclingCyclist_1
      mask Display: image(imread(imagePath));color('white');text(0, 0, ' ID=167\n')
  Male_CyclingCyclist_2 : Subsystem  Tag=WorldObjectSubSystem  InitFcn=UniqueId = '29111';
      mask init: same as W01_Base_Map_cs/Male_CyclingCyclist_1
      mask Display: image(imread(imagePath));color('white');text(0, 0, ' ID=159\n')
  Male_CyclingCyclist_3 : Subsystem  Tag=WorldObjectSubSystem  InitFcn=UniqueId = '29112';
      mask init: same as W01_Base_Map_cs/Male_CyclingCyclist_1
      mask Display: image(imread(imagePath));color('white');text(0, 0, ' ID=160\n')
  Male_CyclingCyclist_4 : Subsystem  Tag=WorldObjectSubSystem  InitFcn=UniqueId = '29113';
      mask init: same as W01_Base_Map_cs/Male_CyclingCyclist_1
      mask Display: image(imread(imagePath));color('white');text(0, 0, ' ID=161\n')
  Male_CyclingCyclist_5 : Subsystem  Tag=WorldObjectSubSystem  InitFcn=UniqueId = '29114';
      mask init: same as W01_Base_Map_cs/Male_CyclingCyclist_1
      mask Display: image(imread(imagePath));color('white');text(0, 0, ' ID=162\n')
  Male_CyclingCyclist_6 : Subsystem  Tag=WorldObjectSubSystem  InitFcn=UniqueId = '29115';
      mask init: same as W01_Base_Map_cs/Male_CyclingCyclist_1
      mask Display: image(imread(imagePath));color('white');text(0, 0, ' ID=163\n')
  Male_CyclingCyclist_7 : Subsystem  Tag=WorldObjectSubSystem  InitFcn=UniqueId = '29116';
      mask init: same as W01_Base_Map_cs/Male_CyclingCyclist_1
      mask Display: image(imread(imagePath));color('white');text(0, 0, ' ID=164\n')
  Male_CyclingCyclist_8 : Subsystem  Tag=WorldObjectSubSystem  InitFcn=UniqueId = '29117';
      mask init: same as W01_Base_Map_cs/Male_CyclingCyclist_1
      mask Display: image(imread(imagePath));color('white');text(0, 0, ' ID=165\n')
  Male_CyclingCyclist_9 : Subsystem  Tag=WorldObjectSubSystem  InitFcn=UniqueId = '29118';
      mask init: same as W01_Base_Map_cs/Male_CyclingCyclist_1
      mask Display: image(imread(imagePath));color('white');text(0, 0, ' ID=166\n')
  Male_LargeShoulderSuitcase_1 : Subsystem  Tag=WorldObjectSubSystem  InitFcn=UniqueId = '28604';
      mask init:
      | modelPath = GenericModelHelper.getGenericModelFilePath('ModelDepo','Humans\Male_LargeShoulderSuitcase\Male_LargeShoulderSuitcase.pgmb','55ce2ddf27d79dd209e54d76723bb4a0');imagePath = GenericModelHelper.getCompilationPicture(modelPath, 'Male_LargeShoulderSuitcase.png');
      mask Display: image(imread(imagePath));color('white');text(0, 0, ' ID=117\n')
  Male_Old_White_WithStick_1 : Subsystem  Tag=WorldObjectSubSystem  InitFcn=UniqueId = '29054';
      mask init:
      | modelPath = GenericModelHelper.getGenericModelFilePath('ModelDepo','Humans\MaleOld_wStick\MaleOld_wStick.pgmb','72c4e892f653051a1b5626fd66af8f53');imagePath = GenericModelHelper.getCompilationPicture(modelPath, 'MaleOld_Stick.png');
      mask Display: image(imread(imagePath));color('white');text(0, 0, ' ID=130\n')
  Male_Old_White_WithWalkerWithWheels_1 : Subsystem  Tag=WorldObjectSubSystem  InitFcn=UniqueId = '29060';
      mask init:
      | modelPath = GenericModelHelper.getGenericModelFilePath('ModelDepo','Humans\MaleOld_wRollator\MaleOld_wRollator.pgmb','e66e6b4c6dc3e63e11784c58b6ebe541');imagePath = GenericModelHelper.getCompilationPicture(modelPath, 'MaleOld_Rollator.png');
      mask Display: image(imread(imagePath));color('white');text(0, 0, ' ID=136\n')
  Male_Old_White_WithWalker_1 : Subsystem  Tag=WorldObjectSubSystem  InitFcn=UniqueId = '29059';
      mask init:
      | modelPath = GenericModelHelper.getGenericModelFilePath('ModelDepo','Humans\MaleOld_wWalker\MaleOld_wWalker.pgmb','db567ba73fe418ec87d535b1a23a1fbb');imagePath = GenericModelHelper.getCompilationPicture(modelPath, 'MaleOld_Walker.png');
      mask Display: image(imread(imagePath));color('white');text(0, 0, ' ID=135\n')
  Male_Overweight_1 : Subsystem  Tag=WorldObjectSubSystem  InitFcn=UniqueId = '29055';
      mask init:
      | modelPath = GenericModelHelper.getGenericModelFilePath('ModelDepo','Humans\MaleOverweight\Male_Overweight.pgmb','4c1ee2af6dc63dfe27bf35d056d07c62');imagePath = GenericModelHelper.getCompilationPicture(modelPath, 'MaleOverweight.png');
      mask Display: image(imread(imagePath));color('white');text(0, 0, ' ID=131\n')
  Male_ShoppingBag_1 : Subsystem  Tag=WorldObjectSubSystem  InitFcn=UniqueId = '28603';
      mask init:
      | modelPath = GenericModelHelper.getGenericModelFilePath('ModelDepo','Humans\Male_ShoppingBag\Male_ShoppingBag.pgmb','4b53be81be5f7e7c45a47de211a4e883');imagePath = GenericModelHelper.getCompilationPicture(modelPath, 'Male_ShoppingBag.png');
      mask Display: image(imread(imagePath));color('white');text(0, 0, ' ID=116\n')
  Male_wBackpack_1 : Subsystem  Tag=WorldObjectSubSystem  InitFcn=UniqueId = '28602';
      mask init:
      | modelPath = GenericModelHelper.getGenericModelFilePath('ModelDepo','Humans\MaleBackpack\Male_wBackpack.pgmb','4989abe8b0654fc75f34bfe941ecf3b1');imagePath = GenericModelHelper.getCompilationPicture(modelPath, 'MaleBackpack.png');
      mask Display: image(imread(imagePath));color('white');text(0, 0, ' ID=115\n')
  Male_wLargeBackpack_1 : Subsystem  Tag=WorldObjectSubSystem  InitFcn=UniqueId = '28601';
      mask init:
      | modelPath = GenericModelHelper.getGenericModelFilePath('ModelDepo','Humans\Male_wLargeBackpack\Male_wLargeBackpack.pgmb','6f019451e42e74902a1dfd7498a02865');imagePath = GenericModelHelper.getCompilationPicture(modelPath, 'Male_wLargeBackpack.png');
      mask Display: image(imread(imagePath));color('white');text(0, 0, ' ID=109\n')
  Male_wLongCoat_1 : Subsystem  Tag=WorldObjectSubSystem  InitFcn=UniqueId = '28605';
      mask init:
      | modelPath = GenericModelHelper.getGenericModelFilePath('ModelDepo','Humans\Male_wLongCoat\Male_wLongCoat.pgmb','361d79c83e3106abbb87b62747c5330c');imagePath = GenericModelHelper.getCompilationPicture(modelPath, 'Male_wLongCoat.png');
      mask Display: image(imread(imagePath));color('white');text(0, 0, ' ID=118\n')
  Male_wSuit_1 : Subsystem  Tag=WorldObjectSubSystem  InitFcn=UniqueId = '29056';
      mask init:
      | modelPath = GenericModelHelper.getGenericModelFilePath('ModelDepo','Humans\MaleSuit\Male_wSuit.pgmb','6afb05019f13b11b83c2e34bdb540507');imagePath = GenericModelHelper.getCompilationPicture(modelPath, 'MaleSuit.png');
      mask Display: image(imread(imagePath));color('white');text(0, 0, ' ID=132\n')
  Man_250_1 : Subsystem  Tag=WorldObjectSubSystem  InitFcn=UniqueId = '29058';
      mask init:
      | modelPath = GenericModelHelper.getGenericModelFilePath('ModelDepo','Humans\Man_250\Man_250.pgmb','d552687b60780d871f7a0144e7f81878');imagePath = GenericModelHelper.getCompilationPicture(modelPath, 'Man_250.png');
      mask Display: image(imread(imagePath));color('white');text(0, 0, ' ID=134\n')
  Mazda_RX8_Coupe_1 : Subsystem  Tag=WorldObjectSubSystem  InitFcn=UniqueId = '29070';
      mask init:
      | modelPath = GenericModelHelper.getGenericModelFilePath('ModelDepo','Vehicles\Mazda_RX8\Mazda_RX8.pgmb','1e55a2e40efa576b7f4fb93bae35d605');imagePath = GenericModelHelper.getCompilationPicture(modelPath, 'Mazda_RX8_HighPoly.png');
      mask Display: image(imread(imagePath));color('white');text(0, 0, ' ID=146\n')
  PointCloudSensor_1 : Subsystem  Tag=sensor/PointCloudInport  Priority=30  mask(PreScan Source Block: Point Cloud Sensor){}
      mask help: The Point Cloud Sensor provides XYZ positions relative to the sensor
      settings: OpenFcn=open_system([gcb '/Sensor'],'mask')
      mask Help: eval('openHelp(6400)')
      mask Display: image(imread('PointCloudSensorSL.png'))
  PointCloudSensor_2 : Subsystem  Tag=sensor/PointCloudInport  Priority=30  mask(PreScan Source Block: Point Cloud Sensor){}
      mask help: The Point Cloud Sensor provides XYZ positions relative to the sensor
      settings: OpenFcn=open_system([gcb '/Sensor'],'mask')
      mask Help: eval('openHelp(6400)')
      mask Display: image(imread('PointCloudSensorSL.png'))
  PointCloudSensor_3 : Subsystem  Tag=sensor/PointCloudInport  Priority=30  mask(PreScan Source Block: Point Cloud Sensor){}
      mask help: The Point Cloud Sensor provides XYZ positions relative to the sensor
      settings: OpenFcn=open_system([gcb '/Sensor'],'mask')
      mask Help: eval('openHelp(6400)')
      mask Display: image(imread('PointCloudSensorSL.png'))
  PointCloudSensor_4 : Subsystem  Tag=sensor/PointCloudInport  Priority=30  mask(PreScan Source Block: Point Cloud Sensor){}
      mask help: The Point Cloud Sensor provides XYZ positions relative to the sensor
      settings: OpenFcn=open_system([gcb '/Sensor'],'mask')
      mask Help: eval('openHelp(6400)')
      mask Display: image(imread('PointCloudSensorSL.png'))
  PreScanTerminator : Subsystem  Tag=PreScanTerminator  Priority=999  LoadFcn=load PrescanTerminatorData  mask(PreScan Simulation Terminator){TimeStep=1/20}
      mask prompts: TimeStep "Upload Period [s]"
      mask help: Please do not remove this block from the compilation sheet as it connects the model to the PreScan environment.
      mask Help: eval('openHelp(812)')
      mask Display: image(imread('prescanlogo.ico'))
  Radar_1 : Subsystem  Tag=sensor/Radar  Priority=30  LoadFcn=load('PrescanScannerSensorData.mat');load('PrescanScannerSensorMessage.mat')  mask(PreScan Source Block: Radar Sensor){}
      mask help: The Radar Sensor is a detailed sensor based on a physical radar model that includes Antenna GAIN Maps (AGM) and atmospheric attenuation. For more information, please click Help.
      settings: OpenFcn=open_system([gcb '/Sensor'],'mask')
      mask Help: eval('openHelp(1464)')
      mask Display: image(imread('Radar.png'))
  Roewe_550_S_Sedan_1 : Subsystem  Tag=WorldObjectSubSystem  InitFcn=UniqueId = '29071';
      mask init:
      | modelPath = GenericModelHelper.getGenericModelFilePath('ModelDepo','Vehicles\Roewe_550_S\Roewe_550_S.pgmb','82c18f6c16b5efd393844e3f545cde09');imagePath = GenericModelHelper.getCompilationPicture(modelPath, 'Roewe_550_S_HighPoly.png');
      mask Display: image(imread(imagePath));color('white');text(0, 0, ' ID=147\n')
  SELF_Audi_A3_1 : Subsystem  Tag=sensor/SelfPort  Priority=30  LoadFcn=load('PreScanSelfSensorData.mat')  mask(PreScan Source Block: SELF){}
      mask help: The SELF port shows (state) information of the actor itself. The outputs are position in the experiment's axis system and the GPS coordinates, and the object's absolute velocity and compass heading. For more information, please click Help.
      settings: OpenFcn=open_system([gcb '/Sensor'],'mask')
      mask Help: eval('openHelp(462)')
      mask Display: image(imread('GPS.png'))
  SELF_Audi_A3_2 : Subsystem  Tag=sensor/SelfPort  Priority=30  LoadFcn=load('PreScanSelfSensorData.mat')  mask(PreScan Source Block: SELF){}
      mask help: The SELF port shows (state) information of the actor itself. The outputs are position in the experiment's axis system and the GPS coordinates, and the object's absolute velocity and compass heading. For more information, please click Help.
      settings: OpenFcn=open_system([gcb '/Sensor'],'mask')
      mask Help: eval('openHelp(462)')
      mask Display: image(imread('GPS.png'))
  SELF_Audi_A8_Sedan_2 : Subsystem  Tag=sensor/SelfPort  Priority=30  LoadFcn=load('PreScanSelfSensorData.mat')  mask(PreScan Source Block: SELF){}
      mask help: The SELF port shows (state) information of the actor itself. The outputs are position in the experiment's axis system and the GPS coordinates, and the object's absolute velocity and compass heading. For more information, please click Help.
      settings: OpenFcn=open_system([gcb '/Sensor'],'mask')
      mask Help: eval('openHelp(462)')
      mask Display: image(imread('GPS.png'))
  SELF_BMW_X5_SUV_1 : Subsystem  Tag=sensor/SelfPort  Priority=30  LoadFcn=load('PreScanSelfSensorData.mat')  mask(PreScan Source Block: SELF){}
      mask help: The SELF port shows (state) information of the actor itself. The outputs are position in the experiment's axis system and the GPS coordinates, and the object's absolute velocity and compass heading. For more information, please click Help.
      settings: OpenFcn=open_system([gcb '/Sensor'],'mask')
      mask Help: eval('openHelp(462)')
      mask Display: image(imread('GPS.png'))
  SELF_BMW_Z3_Convertible_1 : Subsystem  Tag=sensor/SelfPort  Priority=30  LoadFcn=load('PreScanSelfSensorData.mat')  mask(PreScan Source Block: SELF){}
      mask help: The SELF port shows (state) information of the actor itself. The outputs are position in the experiment's axis system and the GPS coordinates, and the object's absolute velocity and compass heading. For more information, please click Help.
      settings: OpenFcn=open_system([gcb '/Sensor'],'mask')
      mask Help: eval('openHelp(462)')
      mask Display: image(imread('GPS.png'))
  SELF_Boy_150_1 : Subsystem  Tag=sensor/SelfPort  Priority=30  LoadFcn=load('PreScanSelfSensorData.mat')  mask(PreScan Source Block: SELF){}
      mask help: The SELF port shows (state) information of the actor itself. The outputs are position in the experiment's axis system and the GPS coordinates, and the object's absolute velocity and compass heading. For more information, please click Help.
      settings: OpenFcn=open_system([gcb '/Sensor'],'mask')
      mask Help: eval('openHelp(462)')
      mask Display: image(imread('GPS.png'))
  SELF_Child_Overweight_1 : Subsystem  Tag=sensor/SelfPort  Priority=30  LoadFcn=load('PreScanSelfSensorData.mat')  mask(PreScan Source Block: SELF){}
      mask help: The SELF port shows (state) information of the actor itself. The outputs are position in the experiment's axis system and the GPS coordinates, and the object's absolute velocity and compass heading. For more information, please click Help.
      settings: OpenFcn=open_system([gcb '/Sensor'],'mask')
      mask Help: eval('openHelp(462)')
      mask Display: image(imread('GPS.png'))
  SELF_Citroen_C3_Hatchback_2 : Subsystem  Tag=sensor/SelfPort  Priority=30  LoadFcn=load('PreScanSelfSensorData.mat')  mask(PreScan Source Block: SELF){}
      mask help: The SELF port shows (state) information of the actor itself. The outputs are position in the experiment's axis system and the GPS coordinates, and the object's absolute velocity and compass heading. For more information, please click Help.
      settings: OpenFcn=open_system([gcb '/Sensor'],'mask')
      mask Help: eval('openHelp(462)')
      mask Display: image(imread('GPS.png'))
  SELF_Citroen_C3_Hatchback_3 : Subsystem  Tag=sensor/SelfPort  Priority=30  LoadFcn=load('PreScanSelfSensorData.mat')  mask(PreScan Source Block: SELF){}
      mask help: The SELF port shows (state) information of the actor itself. The outputs are position in the experiment's axis system and the GPS coordinates, and the object's absolute velocity and compass heading. For more information, please click Help.
      settings: OpenFcn=open_system([gcb '/Sensor'],'mask')
      mask Help: eval('openHelp(462)')
      mask Display: image(imread('GPS.png'))
  SELF_Female_Overweight_1 : Subsystem  Tag=sensor/SelfPort  Priority=30  LoadFcn=load('PreScanSelfSensorData.mat')  mask(PreScan Source Block: SELF){}
      mask help: The SELF port shows (state) information of the actor itself. The outputs are position in the experiment's axis system and the GPS coordinates, and the object's absolute velocity and compass heading. For more information, please click Help.
      settings: OpenFcn=open_system([gcb '/Sensor'],'mask')
      mask Help: eval('openHelp(462)')
      mask Display: image(imread('GPS.png'))
  SELF_Female_Regular_1 : Subsystem  Tag=sensor/SelfPort  Priority=30  LoadFcn=load('PreScanSelfSensorData.mat')  mask(PreScan Source Block: SELF){}
      mask help: The SELF port shows (state) information of the actor itself. The outputs are position in the experiment's axis system and the GPS coordinates, and the object's absolute velocity and compass heading. For more information, please click Help.
      settings: OpenFcn=open_system([gcb '/Sensor'],'mask')
      mask Help: eval('openHelp(462)')
      mask Display: image(imread('GPS.png'))
  SELF_Female_wBuggy_1 : Subsystem  Tag=sensor/SelfPort  Priority=30  LoadFcn=load('PreScanSelfSensorData.mat')  mask(PreScan Source Block: SELF){}
      mask help: The SELF port shows (state) information of the actor itself. The outputs are position in the experiment's axis system and the GPS coordinates, and the object's absolute velocity and compass heading. For more information, please click Help.
      settings: OpenFcn=open_system([gcb '/Sensor'],'mask')
      mask Help: eval('openHelp(462)')
      mask Display: image(imread('GPS.png'))
  SELF_Female_wLongCoat_1 : Subsystem  Tag=sensor/SelfPort  Priority=30  LoadFcn=load('PreScanSelfSensorData.mat')  mask(PreScan Source Block: SELF){}
      mask help: The SELF port shows (state) information of the actor itself. The outputs are position in the experiment's axis system and the GPS coordinates, and the object's absolute velocity and compass heading. For more information, please click Help.
      settings: OpenFcn=open_system([gcb '/Sensor'],'mask')
      mask Help: eval('openHelp(462)')
      mask Display: image(imread('GPS.png'))
  SELF_Female_wRaincoat_1 : Subsystem  Tag=sensor/SelfPort  Priority=30  LoadFcn=load('PreScanSelfSensorData.mat')  mask(PreScan Source Block: SELF){}
      mask help: The SELF port shows (state) information of the actor itself. The outputs are position in the experiment's axis system and the GPS coordinates, and the object's absolute velocity and compass heading. For more information, please click Help.
      settings: OpenFcn=open_system([gcb '/Sensor'],'mask')
      mask Help: eval('openHelp(462)')
      mask Display: image(imread('GPS.png'))
  SELF_Fiat_Bravo_Hatchback_1 : Subsystem  Tag=sensor/SelfPort  Priority=30  LoadFcn=load('PreScanSelfSensorData.mat')  mask(PreScan Source Block: SELF){}
      mask help: The SELF port shows (state) information of the actor itself. The outputs are position in the experiment's axis system and the GPS coordinates, and the object's absolute velocity and compass heading. For more information, please click Help.
      settings: OpenFcn=open_system([gcb '/Sensor'],'mask')
      mask Help: eval('openHelp(462)')
      mask Display: image(imread('GPS.png'))
  SELF_Ford_Fiesta_Hatchback_2 : Subsystem  Tag=sensor/SelfPort  Priority=30  LoadFcn=load('PreScanSelfSensorData.mat')  mask(PreScan Source Block: SELF){}
      mask help: The SELF port shows (state) information of the actor itself. The outputs are position in the experiment's axis system and the GPS coordinates, and the object's absolute velocity and compass heading. For more information, please click Help.
      settings: OpenFcn=open_system([gcb '/Sensor'],'mask')
      mask Help: eval('openHelp(462)')
      mask Display: image(imread('GPS.png'))
  SELF_Ford_Focus_Stationwagon_1 : Subsystem  Tag=sensor/SelfPort  Priority=30  LoadFcn=load('PreScanSelfSensorData.mat')  mask(PreScan Source Block: SELF){}
      mask help: The SELF port shows (state) information of the actor itself. The outputs are position in the experiment's axis system and the GPS coordinates, and the object's absolute velocity and compass heading. For more information, please click Help.
      settings: OpenFcn=open_system([gcb '/Sensor'],'mask')
      mask Help: eval('openHelp(462)')
      mask Display: image(imread('GPS.png'))
  SELF_Honda_Pan_European_Motorcycle_With_Driver_1 : Subsystem  Tag=sensor/SelfPort  Priority=30  LoadFcn=load('PreScanSelfSensorData.mat')  mask(PreScan Source Block: SELF){}
      mask help: The SELF port shows (state) information of the actor itself. The outputs are position in the experiment's axis system and the GPS coordinates, and the object's absolute velocity and compass heading. For more information, please click Help.
      settings: OpenFcn=open_system([gcb '/Sensor'],'mask')
      mask Help: eval('openHelp(462)')
      mask Display: image(imread('GPS.png'))
  SELF_Honda_Pan_European_Motorcycle_With_Driver_2 : Subsystem  Tag=sensor/SelfPort  Priority=30  LoadFcn=load('PreScanSelfSensorData.mat')  mask(PreScan Source Block: SELF){}
      mask help: The SELF port shows (state) information of the actor itself. The outputs are position in the experiment's axis system and the GPS coordinates, and the object's absolute velocity and compass heading. For more information, please click Help.
      settings: OpenFcn=open_system([gcb '/Sensor'],'mask')
      mask Help: eval('openHelp(462)')
      mask Display: image(imread('GPS.png'))
  SELF_Lexus_GS_450h_F_Sport_Sedan_1 : Subsystem  Tag=sensor/SelfPort  Priority=30  LoadFcn=load('PreScanSelfSensorData.mat')  mask(PreScan Source Block: SELF){}
      mask help: The SELF port shows (state) information of the actor itself. The outputs are position in the experiment's axis system and the GPS coordinates, and the object's absolute velocity and compass heading. For more information, please click Help.
      settings: OpenFcn=open_system([gcb '/Sensor'],'mask')
      mask Help: eval('openHelp(462)')
      mask Display: image(imread('GPS.png'))
  SELF_Lexus_LS_600h_F_Sport_1 : Subsystem  Tag=sensor/SelfPort  Priority=30  LoadFcn=load('PreScanSelfSensorData.mat')  mask(PreScan Source Block: SELF){}
      mask help: The SELF port shows (state) information of the actor itself. The outputs are position in the experiment's axis system and the GPS coordinates, and the object's absolute velocity and compass heading. For more information, please click Help.
      settings: OpenFcn=open_system([gcb '/Sensor'],'mask')
      mask Help: eval('openHelp(462)')
      mask Display: image(imread('GPS.png'))
  SELF_Male_200_1 : Subsystem  Tag=sensor/SelfPort  Priority=30  LoadFcn=load('PreScanSelfSensorData.mat')  mask(PreScan Source Block: SELF){}
      mask help: The SELF port shows (state) information of the actor itself. The outputs are position in the experiment's axis system and the GPS coordinates, and the object's absolute velocity and compass heading. For more information, please click Help.
      settings: OpenFcn=open_system([gcb '/Sensor'],'mask')
      mask Help: eval('openHelp(462)')
      mask Display: image(imread('GPS.png'))
  SELF_Male_African_1 : Subsystem  Tag=sensor/SelfPort  Priority=30  LoadFcn=load('PreScanSelfSensorData.mat')  mask(PreScan Source Block: SELF){}
      mask help: The SELF port shows (state) information of the actor itself. The outputs are position in the experiment's axis system and the GPS coordinates, and the object's absolute velocity and compass heading. For more information, please click Help.
      settings: OpenFcn=open_system([gcb '/Sensor'],'mask')
      mask Help: eval('openHelp(462)')
      mask Display: image(imread('GPS.png'))
  SELF_Male_CyclingCyclist_1 : Subsystem  Tag=sensor/SelfPort  Priority=30  LoadFcn=load('PreScanSelfSensorData.mat')  mask(PreScan Source Block: SELF){}
      mask help: The SELF port shows (state) information of the actor itself. The outputs are position in the experiment's axis system and the GPS coordinates, and the object's absolute velocity and compass heading. For more information, please click Help.
      settings: OpenFcn=open_system([gcb '/Sensor'],'mask')
      mask Help: eval('openHelp(462)')
      mask Display: image(imread('GPS.png'))
  SELF_Male_CyclingCyclist_10 : Subsystem  Tag=sensor/SelfPort  Priority=30  LoadFcn=load('PreScanSelfSensorData.mat')  mask(PreScan Source Block: SELF){}
      mask help: The SELF port shows (state) information of the actor itself. The outputs are position in the experiment's axis system and the GPS coordinates, and the object's absolute velocity and compass heading. For more information, please click Help.
      settings: OpenFcn=open_system([gcb '/Sensor'],'mask')
      mask Help: eval('openHelp(462)')
      mask Display: image(imread('GPS.png'))
  SELF_Male_CyclingCyclist_2 : Subsystem  Tag=sensor/SelfPort  Priority=30  LoadFcn=load('PreScanSelfSensorData.mat')  mask(PreScan Source Block: SELF){}
      mask help: The SELF port shows (state) information of the actor itself. The outputs are position in the experiment's axis system and the GPS coordinates, and the object's absolute velocity and compass heading. For more information, please click Help.
      settings: OpenFcn=open_system([gcb '/Sensor'],'mask')
      mask Help: eval('openHelp(462)')
      mask Display: image(imread('GPS.png'))
  SELF_Male_CyclingCyclist_3 : Subsystem  Tag=sensor/SelfPort  Priority=30  LoadFcn=load('PreScanSelfSensorData.mat')  mask(PreScan Source Block: SELF){}
      mask help: The SELF port shows (state) information of the actor itself. The outputs are position in the experiment's axis system and the GPS coordinates, and the object's absolute velocity and compass heading. For more information, please click Help.
      settings: OpenFcn=open_system([gcb '/Sensor'],'mask')
      mask Help: eval('openHelp(462)')
      mask Display: image(imread('GPS.png'))
  SELF_Male_CyclingCyclist_4 : Subsystem  Tag=sensor/SelfPort  Priority=30  LoadFcn=load('PreScanSelfSensorData.mat')  mask(PreScan Source Block: SELF){}
      mask help: The SELF port shows (state) information of the actor itself. The outputs are position in the experiment's axis system and the GPS coordinates, and the object's absolute velocity and compass heading. For more information, please click Help.
      settings: OpenFcn=open_system([gcb '/Sensor'],'mask')
      mask Help: eval('openHelp(462)')
      mask Display: image(imread('GPS.png'))
  SELF_Male_CyclingCyclist_5 : Subsystem  Tag=sensor/SelfPort  Priority=30  LoadFcn=load('PreScanSelfSensorData.mat')  mask(PreScan Source Block: SELF){}
      mask help: The SELF port shows (state) information of the actor itself. The outputs are position in the experiment's axis system and the GPS coordinates, and the object's absolute velocity and compass heading. For more information, please click Help.
      settings: OpenFcn=open_system([gcb '/Sensor'],'mask')
      mask Help: eval('openHelp(462)')
      mask Display: image(imread('GPS.png'))
  SELF_Male_CyclingCyclist_6 : Subsystem  Tag=sensor/SelfPort  Priority=30  LoadFcn=load('PreScanSelfSensorData.mat')  mask(PreScan Source Block: SELF){}
      mask help: The SELF port shows (state) information of the actor itself. The outputs are position in the experiment's axis system and the GPS coordinates, and the object's absolute velocity and compass heading. For more information, please click Help.
      settings: OpenFcn=open_system([gcb '/Sensor'],'mask')
      mask Help: eval('openHelp(462)')
      mask Display: image(imread('GPS.png'))
  SELF_Male_CyclingCyclist_7 : Subsystem  Tag=sensor/SelfPort  Priority=30  LoadFcn=load('PreScanSelfSensorData.mat')  mask(PreScan Source Block: SELF){}
      mask help: The SELF port shows (state) information of the actor itself. The outputs are position in the experiment's axis system and the GPS coordinates, and the object's absolute velocity and compass heading. For more information, please click Help.
      settings: OpenFcn=open_system([gcb '/Sensor'],'mask')
      mask Help: eval('openHelp(462)')
      mask Display: image(imread('GPS.png'))
  SELF_Male_CyclingCyclist_8 : Subsystem  Tag=sensor/SelfPort  Priority=30  LoadFcn=load('PreScanSelfSensorData.mat')  mask(PreScan Source Block: SELF){}
      mask help: The SELF port shows (state) information of the actor itself. The outputs are position in the experiment's axis system and the GPS coordinates, and the object's absolute velocity and compass heading. For more information, please click Help.
      settings: OpenFcn=open_system([gcb '/Sensor'],'mask')
      mask Help: eval('openHelp(462)')
      mask Display: image(imread('GPS.png'))
  SELF_Male_CyclingCyclist_9 : Subsystem  Tag=sensor/SelfPort  Priority=30  LoadFcn=load('PreScanSelfSensorData.mat')  mask(PreScan Source Block: SELF){}
      mask help: The SELF port shows (state) information of the actor itself. The outputs are position in the experiment's axis system and the GPS coordinates, and the object's absolute velocity and compass heading. For more information, please click Help.
      settings: OpenFcn=open_system([gcb '/Sensor'],'mask')
      mask Help: eval('openHelp(462)')
      mask Display: image(imread('GPS.png'))
  SELF_Male_LargeShoulderSuitcase_1 : Subsystem  Tag=sensor/SelfPort  Priority=30  LoadFcn=load('PreScanSelfSensorData.mat')  mask(PreScan Source Block: SELF){}
      mask help: The SELF port shows (state) information of the actor itself. The outputs are position in the experiment's axis system and the GPS coordinates, and the object's absolute velocity and compass heading. For more information, please click Help.
      settings: OpenFcn=open_system([gcb '/Sensor'],'mask')
      mask Help: eval('openHelp(462)')
      mask Display: image(imread('GPS.png'))
  SELF_Male_Old_White_WithStick_1 : Subsystem  Tag=sensor/SelfPort  Priority=30  LoadFcn=load('PreScanSelfSensorData.mat')  mask(PreScan Source Block: SELF){}
      mask help: The SELF port shows (state) information of the actor itself. The outputs are position in the experiment's axis system and the GPS coordinates, and the object's absolute velocity and compass heading. For more information, please click Help.
      settings: OpenFcn=open_system([gcb '/Sensor'],'mask')
      mask Help: eval('openHelp(462)')
      mask Display: image(imread('GPS.png'))
  SELF_Male_Old_White_WithWalkerWithWheels_1 : Subsystem  Tag=sensor/SelfPort  Priority=30  LoadFcn=load('PreScanSelfSensorData.mat')  mask(PreScan Source Block: SELF){}
      mask help: The SELF port shows (state) information of the actor itself. The outputs are position in the experiment's axis system and the GPS coordinates, and the object's absolute velocity and compass heading. For more information, please click Help.
      settings: OpenFcn=open_system([gcb '/Sensor'],'mask')
      mask Help: eval('openHelp(462)')
      mask Display: image(imread('GPS.png'))
  SELF_Male_Old_White_WithWalker_1 : Subsystem  Tag=sensor/SelfPort  Priority=30  LoadFcn=load('PreScanSelfSensorData.mat')  mask(PreScan Source Block: SELF){}
      mask help: The SELF port shows (state) information of the actor itself. The outputs are position in the experiment's axis system and the GPS coordinates, and the object's absolute velocity and compass heading. For more information, please click Help.
      settings: OpenFcn=open_system([gcb '/Sensor'],'mask')
      mask Help: eval('openHelp(462)')
      mask Display: image(imread('GPS.png'))
  SELF_Male_Overweight_1 : Subsystem  Tag=sensor/SelfPort  Priority=30  LoadFcn=load('PreScanSelfSensorData.mat')  mask(PreScan Source Block: SELF){}
      mask help: The SELF port shows (state) information of the actor itself. The outputs are position in the experiment's axis system and the GPS coordinates, and the object's absolute velocity and compass heading. For more information, please click Help.
      settings: OpenFcn=open_system([gcb '/Sensor'],'mask')
      mask Help: eval('openHelp(462)')
      mask Display: image(imread('GPS.png'))
  SELF_Male_ShoppingBag_1 : Subsystem  Tag=sensor/SelfPort  Priority=30  LoadFcn=load('PreScanSelfSensorData.mat')  mask(PreScan Source Block: SELF){}
      mask help: The SELF port shows (state) information of the actor itself. The outputs are position in the experiment's axis system and the GPS coordinates, and the object's absolute velocity and compass heading. For more information, please click Help.
      settings: OpenFcn=open_system([gcb '/Sensor'],'mask')
      mask Help: eval('openHelp(462)')
      mask Display: image(imread('GPS.png'))
  SELF_Male_wBackpack_1 : Subsystem  Tag=sensor/SelfPort  Priority=30  LoadFcn=load('PreScanSelfSensorData.mat')  mask(PreScan Source Block: SELF){}
      mask help: The SELF port shows (state) information of the actor itself. The outputs are position in the experiment's axis system and the GPS coordinates, and the object's absolute velocity and compass heading. For more information, please click Help.
      settings: OpenFcn=open_system([gcb '/Sensor'],'mask')
      mask Help: eval('openHelp(462)')
      mask Display: image(imread('GPS.png'))
  SELF_Male_wLargeBackpack_1 : Subsystem  Tag=sensor/SelfPort  Priority=30  LoadFcn=load('PreScanSelfSensorData.mat')  mask(PreScan Source Block: SELF){}
      mask help: The SELF port shows (state) information of the actor itself. The outputs are position in the experiment's axis system and the GPS coordinates, and the object's absolute velocity and compass heading. For more information, please click Help.
      settings: OpenFcn=open_system([gcb '/Sensor'],'mask')
      mask Help: eval('openHelp(462)')
      mask Display: image(imread('GPS.png'))
  SELF_Male_wLongCoat_1 : Subsystem  Tag=sensor/SelfPort  Priority=30  LoadFcn=load('PreScanSelfSensorData.mat')  mask(PreScan Source Block: SELF){}
      mask help: The SELF port shows (state) information of the actor itself. The outputs are position in the experiment's axis system and the GPS coordinates, and the object's absolute velocity and compass heading. For more information, please click Help.
      settings: OpenFcn=open_system([gcb '/Sensor'],'mask')
      mask Help: eval('openHelp(462)')
      mask Display: image(imread('GPS.png'))
  SELF_Male_wSuit_1 : Subsystem  Tag=sensor/SelfPort  Priority=30  LoadFcn=load('PreScanSelfSensorData.mat')  mask(PreScan Source Block: SELF){}
      mask help: The SELF port shows (state) information of the actor itself. The outputs are position in the experiment's axis system and the GPS coordinates, and the object's absolute velocity and compass heading. For more information, please click Help.
      settings: OpenFcn=open_system([gcb '/Sensor'],'mask')
      mask Help: eval('openHelp(462)')
      mask Display: image(imread('GPS.png'))
  SELF_Man_250_1 : Subsystem  Tag=sensor/SelfPort  Priority=30  LoadFcn=load('PreScanSelfSensorData.mat')  mask(PreScan Source Block: SELF){}
      mask help: The SELF port shows (state) information of the actor itself. The outputs are position in the experiment's axis system and the GPS coordinates, and the object's absolute velocity and compass heading. For more information, please click Help.
      settings: OpenFcn=open_system([gcb '/Sensor'],'mask')
      mask Help: eval('openHelp(462)')
      mask Display: image(imread('GPS.png'))
  SELF_Mazda_RX8_Coupe_1 : Subsystem  Tag=sensor/SelfPort  Priority=30  LoadFcn=load('PreScanSelfSensorData.mat')  mask(PreScan Source Block: SELF){}
      mask help: The SELF port shows (state) information of the actor itself. The outputs are position in the experiment's axis system and the GPS coordinates, and the object's absolute velocity and compass heading. For more information, please click Help.
      settings: OpenFcn=open_system([gcb '/Sensor'],'mask')
      mask Help: eval('openHelp(462)')
      mask Display: image(imread('GPS.png'))
  SELF_Roewe_550_S_Sedan_1 : Subsystem  Tag=sensor/SelfPort  Priority=30  LoadFcn=load('PreScanSelfSensorData.mat')  mask(PreScan Source Block: SELF){}
      mask help: The SELF port shows (state) information of the actor itself. The outputs are position in the experiment's axis system and the GPS coordinates, and the object's absolute velocity and compass heading. For more information, please click Help.
      settings: OpenFcn=open_system([gcb '/Sensor'],'mask')
      mask Help: eval('openHelp(462)')
      mask Display: image(imread('GPS.png'))
  SELF_Sports_Bike_wDriver_1 : Subsystem  Tag=sensor/SelfPort  Priority=30  LoadFcn=load('PreScanSelfSensorData.mat')  mask(PreScan Source Block: SELF){}
      mask help: The SELF port shows (state) information of the actor itself. The outputs are position in the experiment's axis system and the GPS coordinates, and the object's absolute velocity and compass heading. For more information, please click Help.
      settings: OpenFcn=open_system([gcb '/Sensor'],'mask')
      mask Help: eval('openHelp(462)')
      mask Display: image(imread('GPS.png'))
  SELF_Sports_Bike_wDriver_2 : Subsystem  Tag=sensor/SelfPort  Priority=30  LoadFcn=load('PreScanSelfSensorData.mat')  mask(PreScan Source Block: SELF){}
      mask help: The SELF port shows (state) information of the actor itself. The outputs are position in the experiment's axis system and the GPS coordinates, and the object's absolute velocity and compass heading. For more information, please click Help.
      settings: OpenFcn=open_system([gcb '/Sensor'],'mask')
      mask Help: eval('openHelp(462)')
      mask Display: image(imread('GPS.png'))
  SELF_Sports_Bike_wDriver_3 : Subsystem  Tag=sensor/SelfPort  Priority=30  LoadFcn=load('PreScanSelfSensorData.mat')  mask(PreScan Source Block: SELF){}
      mask help: The SELF port shows (state) information of the actor itself. The outputs are position in the experiment's axis system and the GPS coordinates, and the object's absolute velocity and compass heading. For more information, please click Help.
      settings: OpenFcn=open_system([gcb '/Sensor'],'mask')
      mask Help: eval('openHelp(462)')
      mask Display: image(imread('GPS.png'))
  SELF_Tesla_Model_3_1 : Subsystem  Tag=sensor/SelfPort  Priority=30  LoadFcn=load('PreScanSelfSensorData.mat')  mask(PreScan Source Block: SELF){}
      mask help: The SELF port shows (state) information of the actor itself. The outputs are position in the experiment's axis system and the GPS coordinates, and the object's absolute velocity and compass heading. For more information, please click Help.
      settings: OpenFcn=open_system([gcb '/Sensor'],'mask')
      mask Help: eval('openHelp(462)')
      mask Display: image(imread('GPS.png'))
  SELF_Toyota_Previa_MPV_1 : Subsystem  Tag=sensor/SelfPort  Priority=30  LoadFcn=load('PreScanSelfSensorData.mat')  mask(PreScan Source Block: SELF){}
      mask help: The SELF port shows (state) information of the actor itself. The outputs are position in the experiment's axis system and the GPS coordinates, and the object's absolute velocity and compass heading. For more information, please click Help.
      settings: OpenFcn=open_system([gcb '/Sensor'],'mask')
      mask Help: eval('openHelp(462)')
      mask Display: image(imread('GPS.png'))
  SELF_Toyota_Prius_Sedan_1 : Subsystem  Tag=sensor/SelfPort  Priority=30  LoadFcn=load('PreScanSelfSensorData.mat')  mask(PreScan Source Block: SELF){}
      mask help: The SELF port shows (state) information of the actor itself. The outputs are position in the experiment's axis system and the GPS coordinates, and the object's absolute velocity and compass heading. For more information, please click Help.
      settings: OpenFcn=open_system([gcb '/Sensor'],'mask')
      mask Help: eval('openHelp(462)')
      mask Display: image(imread('GPS.png'))
  SELF_Toyota_Yaris_Hatchback_1 : Subsystem  Tag=sensor/SelfPort  Priority=30  LoadFcn=load('PreScanSelfSensorData.mat')  mask(PreScan Source Block: SELF){}
      mask help: The SELF port shows (state) information of the actor itself. The outputs are position in the experiment's axis system and the GPS coordinates, and the object's absolute velocity and compass heading. For more information, please click Help.
      settings: OpenFcn=open_system([gcb '/Sensor'],'mask')
      mask Help: eval('openHelp(462)')
      mask Display: image(imread('GPS.png'))
  SELF_Toyota_Yaris_Hatchback_2 : Subsystem  Tag=sensor/SelfPort  Priority=30  LoadFcn=load('PreScanSelfSensorData.mat')  mask(PreScan Source Block: SELF){}
      mask help: The SELF port shows (state) information of the actor itself. The outputs are position in the experiment's axis system and the GPS coordinates, and the object's absolute velocity and compass heading. For more information, please click Help.
      settings: OpenFcn=open_system([gcb '/Sensor'],'mask')
      mask Help: eval('openHelp(462)')
      mask Display: image(imread('GPS.png'))
  SELF_Volvo_XC60_1 : Subsystem  Tag=sensor/SelfPort  Priority=30  LoadFcn=load('PreScanSelfSensorData.mat')  mask(PreScan Source Block: SELF){}
      mask help: The SELF port shows (state) information of the actor itself. The outputs are position in the experiment's axis system and the GPS coordinates, and the object's absolute velocity and compass heading. For more information, please click Help.
      settings: OpenFcn=open_system([gcb '/Sensor'],'mask')
      mask Help: eval('openHelp(462)')
      mask Display: image(imread('GPS.png'))
  SELF_Wuling_Hongguang_1 : Subsystem  Tag=sensor/SelfPort  Priority=30  LoadFcn=load('PreScanSelfSensorData.mat')  mask(PreScan Source Block: SELF){}
      mask help: The SELF port shows (state) information of the actor itself. The outputs are position in the experiment's axis system and the GPS coordinates, and the object's absolute velocity and compass heading. For more information, please click Help.
      settings: OpenFcn=open_system([gcb '/Sensor'],'mask')
      mask Help: eval('openHelp(462)')
      mask Display: image(imread('GPS.png'))
  STATE_Audi_A3_1_bus : Subsystem  Tag=actuator/StatePort  Priority=0  LoadFcn=load('PreScanStateActuatorData.mat')  mask(PreScan Sink Block: State){}
      mask help: The Actor State contains a vector signal of size (9x1), containing the following signals: - Position (x,y,z) [m] - Velocity (vx,vy,vz) [m/s] - Angles (Roll, Pitch, Yaw) [rad] The Actor state is defined in the global axis system. The state is superponed on the Initial position defined in the GUI. For more information, please click Help.
      settings: OpenFcn=open_system([gcb '/Actuator'],'mask')
      mask Help: eval('openHelp(222)')
      mask Display: image(imread('State.png'))
  STATE_Audi_A3_2_bus : Subsystem  Tag=actuator/StatePort  Priority=0  LoadFcn=load('PreScanStateActuatorData.mat')  mask(PreScan Sink Block: State){}
      mask help: The Actor State contains a vector signal of size (9x1), containing the following signals: - Position (x,y,z) [m] - Velocity (vx,vy,vz) [m/s] - Angles (Roll, Pitch, Yaw) [rad] The Actor state is defined in the global axis system. The state is superponed on the Initial position defined in the GUI. For more information, please click Help.
      settings: OpenFcn=open_system([gcb '/Actuator'],'mask')
      mask Help: eval('openHelp(222)')
      mask Display: image(imread('State.png'))
  STATE_Audi_A8_Sedan_2_bus : Subsystem  Tag=actuator/StatePort  Priority=0  LoadFcn=load('PreScanStateActuatorData.mat')  mask(PreScan Sink Block: State){}
      mask help: The Actor State contains a vector signal of size (9x1), containing the following signals: - Position (x,y,z) [m] - Velocity (vx,vy,vz) [m/s] - Angles (Roll, Pitch, Yaw) [rad] The Actor state is defined in the global axis system. The state is superponed on the Initial position defined in the GUI. For more information, please click Help.
      settings: OpenFcn=open_system([gcb '/Actuator'],'mask')
      mask Help: eval('openHelp(222)')
      mask Display: image(imread('State.png'))
  STATE_BMW_X5_SUV_1_bus : Subsystem  Tag=actuator/StatePort  Priority=0  LoadFcn=load('PreScanStateActuatorData.mat')  mask(PreScan Sink Block: State){}
      mask help: The Actor State contains a vector signal of size (9x1), containing the following signals: - Position (x,y,z) [m] - Velocity (vx,vy,vz) [m/s] - Angles (Roll, Pitch, Yaw) [rad] The Actor state is defined in the global axis system. The state is superponed on the Initial position defined in the GUI. For more information, please click Help.
      settings: OpenFcn=open_system([gcb '/Actuator'],'mask')
      mask Help: eval('openHelp(222)')
      mask Display: image(imread('State.png'))
  STATE_BMW_Z3_Convertible_1_bus : Subsystem  Tag=actuator/StatePort  Priority=0  LoadFcn=load('PreScanStateActuatorData.mat')  mask(PreScan Sink Block: State){}
      mask help: The Actor State contains a vector signal of size (9x1), containing the following signals: - Position (x,y,z) [m] - Velocity (vx,vy,vz) [m/s] - Angles (Roll, Pitch, Yaw) [rad] The Actor state is defined in the global axis system. The state is superponed on the Initial position defined in the GUI. For more information, please click Help.
      settings: OpenFcn=open_system([gcb '/Actuator'],'mask')
      mask Help: eval('openHelp(222)')
      mask Display: image(imread('State.png'))
  STATE_Boy_150_1_bus : Subsystem  Tag=actuator/StatePort  Priority=0  LoadFcn=load('PreScanStateActuatorData.mat')  mask(PreScan Sink Block: State){}
      mask help: The Actor State contains a vector signal of size (9x1), containing the following signals: - Position (x,y,z) [m] - Velocity (vx,vy,vz) [m/s] - Angles (Roll, Pitch, Yaw) [rad] The Actor state is defined in the global axis system. The state is superponed on the Initial position defined in the GUI. For more information, please click Help.
      settings: OpenFcn=open_system([gcb '/Actuator'],'mask')
      mask Help: eval('openHelp(222)')
      mask Display: image(imread('State.png'))
  STATE_Child_Overweight_1_bus : Subsystem  Tag=actuator/StatePort  Priority=0  LoadFcn=load('PreScanStateActuatorData.mat')  mask(PreScan Sink Block: State){}
      mask help: The Actor State contains a vector signal of size (9x1), containing the following signals: - Position (x,y,z) [m] - Velocity (vx,vy,vz) [m/s] - Angles (Roll, Pitch, Yaw) [rad] The Actor state is defined in the global axis system. The state is superponed on the Initial position defined in the GUI. For more information, please click Help.
      settings: OpenFcn=open_system([gcb '/Actuator'],'mask')
      mask Help: eval('openHelp(222)')
      mask Display: image(imread('State.png'))
  STATE_Citroen_C3_Hatchback_2_bus : Subsystem  Tag=actuator/StatePort  Priority=0  LoadFcn=load('PreScanStateActuatorData.mat')  mask(PreScan Sink Block: State){}
      mask help: The Actor State contains a vector signal of size (9x1), containing the following signals: - Position (x,y,z) [m] - Velocity (vx,vy,vz) [m/s] - Angles (Roll, Pitch, Yaw) [rad] The Actor state is defined in the global axis system. The state is superponed on the Initial position defined in the GUI. For more information, please click Help.
      settings: OpenFcn=open_system([gcb '/Actuator'],'mask')
      mask Help: eval('openHelp(222)')
      mask Display: image(imread('State.png'))
  STATE_Citroen_C3_Hatchback_3_bus : Subsystem  Tag=actuator/StatePort  Priority=0  LoadFcn=load('PreScanStateActuatorData.mat')  mask(PreScan Sink Block: State){}
      mask help: The Actor State contains a vector signal of size (9x1), containing the following signals: - Position (x,y,z) [m] - Velocity (vx,vy,vz) [m/s] - Angles (Roll, Pitch, Yaw) [rad] The Actor state is defined in the global axis system. The state is superponed on the Initial position defined in the GUI. For more information, please click Help.
      settings: OpenFcn=open_system([gcb '/Actuator'],'mask')
      mask Help: eval('openHelp(222)')
      mask Display: image(imread('State.png'))
  STATE_Female_Overweight_1_bus : Subsystem  Tag=actuator/StatePort  Priority=0  LoadFcn=load('PreScanStateActuatorData.mat')  mask(PreScan Sink Block: State){}
      mask help: The Actor State contains a vector signal of size (9x1), containing the following signals: - Position (x,y,z) [m] - Velocity (vx,vy,vz) [m/s] - Angles (Roll, Pitch, Yaw) [rad] The Actor state is defined in the global axis system. The state is superponed on the Initial position defined in the GUI. For more information, please click Help.
      settings: OpenFcn=open_system([gcb '/Actuator'],'mask')
      mask Help: eval('openHelp(222)')
      mask Display: image(imread('State.png'))
  STATE_Female_Regular_1_bus : Subsystem  Tag=actuator/StatePort  Priority=0  LoadFcn=load('PreScanStateActuatorData.mat')  mask(PreScan Sink Block: State){}
      mask help: The Actor State contains a vector signal of size (9x1), containing the following signals: - Position (x,y,z) [m] - Velocity (vx,vy,vz) [m/s] - Angles (Roll, Pitch, Yaw) [rad] The Actor state is defined in the global axis system. The state is superponed on the Initial position defined in the GUI. For more information, please click Help.
      settings: OpenFcn=open_system([gcb '/Actuator'],'mask')
      mask Help: eval('openHelp(222)')
      mask Display: image(imread('State.png'))
  STATE_Female_wBuggy_1_bus : Subsystem  Tag=actuator/StatePort  Priority=0  LoadFcn=load('PreScanStateActuatorData.mat')  mask(PreScan Sink Block: State){}
      mask help: The Actor State contains a vector signal of size (9x1), containing the following signals: - Position (x,y,z) [m] - Velocity (vx,vy,vz) [m/s] - Angles (Roll, Pitch, Yaw) [rad] The Actor state is defined in the global axis system. The state is superponed on the Initial position defined in the GUI. For more information, please click Help.
      settings: OpenFcn=open_system([gcb '/Actuator'],'mask')
      mask Help: eval('openHelp(222)')
      mask Display: image(imread('State.png'))
  STATE_Female_wLongCoat_1_bus : Subsystem  Tag=actuator/StatePort  Priority=0  LoadFcn=load('PreScanStateActuatorData.mat')  mask(PreScan Sink Block: State){}
      mask help: The Actor State contains a vector signal of size (9x1), containing the following signals: - Position (x,y,z) [m] - Velocity (vx,vy,vz) [m/s] - Angles (Roll, Pitch, Yaw) [rad] The Actor state is defined in the global axis system. The state is superponed on the Initial position defined in the GUI. For more information, please click Help.
      settings: OpenFcn=open_system([gcb '/Actuator'],'mask')
      mask Help: eval('openHelp(222)')
      mask Display: image(imread('State.png'))
  STATE_Female_wRaincoat_1_bus : Subsystem  Tag=actuator/StatePort  Priority=0  LoadFcn=load('PreScanStateActuatorData.mat')  mask(PreScan Sink Block: State){}
      mask help: The Actor State contains a vector signal of size (9x1), containing the following signals: - Position (x,y,z) [m] - Velocity (vx,vy,vz) [m/s] - Angles (Roll, Pitch, Yaw) [rad] The Actor state is defined in the global axis system. The state is superponed on the Initial position defined in the GUI. For more information, please click Help.
      settings: OpenFcn=open_system([gcb '/Actuator'],'mask')
      mask Help: eval('openHelp(222)')
      mask Display: image(imread('State.png'))
  STATE_Fiat_Bravo_Hatchback_1_bus : Subsystem  Tag=actuator/StatePort  Priority=0  LoadFcn=load('PreScanStateActuatorData.mat')  mask(PreScan Sink Block: State){}
      mask help: The Actor State contains a vector signal of size (9x1), containing the following signals: - Position (x,y,z) [m] - Velocity (vx,vy,vz) [m/s] - Angles (Roll, Pitch, Yaw) [rad] The Actor state is defined in the global axis system. The state is superponed on the Initial position defined in the GUI. For more information, please click Help.
      settings: OpenFcn=open_system([gcb '/Actuator'],'mask')
      mask Help: eval('openHelp(222)')
      mask Display: image(imread('State.png'))
  STATE_Ford_Fiesta_Hatchback_2_bus : Subsystem  Tag=actuator/StatePort  Priority=0  LoadFcn=load('PreScanStateActuatorData.mat')  mask(PreScan Sink Block: State){}
      mask help: The Actor State contains a vector signal of size (9x1), containing the following signals: - Position (x,y,z) [m] - Velocity (vx,vy,vz) [m/s] - Angles (Roll, Pitch, Yaw) [rad] The Actor state is defined in the global axis system. The state is superponed on the Initial position defined in the GUI. For more information, please click Help.
      settings: OpenFcn=open_system([gcb '/Actuator'],'mask')
      mask Help: eval('openHelp(222)')
      mask Display: image(imread('State.png'))
  STATE_Ford_Focus_Stationwagon_1_bus : Subsystem  Tag=actuator/StatePort  Priority=0  LoadFcn=load('PreScanStateActuatorData.mat')  mask(PreScan Sink Block: State){}
      mask help: The Actor State contains a vector signal of size (9x1), containing the following signals: - Position (x,y,z) [m] - Velocity (vx,vy,vz) [m/s] - Angles (Roll, Pitch, Yaw) [rad] The Actor state is defined in the global axis system. The state is superponed on the Initial position defined in the GUI. For more information, please click Help.
      settings: OpenFcn=open_system([gcb '/Actuator'],'mask')
      mask Help: eval('openHelp(222)')
      mask Display: image(imread('State.png'))
  STATE_Honda_Pan_European_Motorcycle_With_Driver_1_bus : Subsystem  Tag=actuator/StatePort  Priority=0  LoadFcn=load('PreScanStateActuatorData.mat')  mask(PreScan Sink Block: State){}
      mask help: The Actor State contains a vector signal of size (9x1), containing the following signals: - Position (x,y,z) [m] - Velocity (vx,vy,vz) [m/s] - Angles (Roll, Pitch, Yaw) [rad] The Actor state is defined in the global axis system. The state is superponed on the Initial position defined in the GUI. For more information, please click Help.
      settings: OpenFcn=open_system([gcb '/Actuator'],'mask')
      mask Help: eval('openHelp(222)')
      mask Display: image(imread('State.png'))
  STATE_Honda_Pan_European_Motorcycle_With_Driver_2_bus : Subsystem  Tag=actuator/StatePort  Priority=0  LoadFcn=load('PreScanStateActuatorData.mat')  mask(PreScan Sink Block: State){}
      mask help: The Actor State contains a vector signal of size (9x1), containing the following signals: - Position (x,y,z) [m] - Velocity (vx,vy,vz) [m/s] - Angles (Roll, Pitch, Yaw) [rad] The Actor state is defined in the global axis system. The state is superponed on the Initial position defined in the GUI. For more information, please click Help.
      settings: OpenFcn=open_system([gcb '/Actuator'],'mask')
      mask Help: eval('openHelp(222)')
      mask Display: image(imread('State.png'))
  STATE_Lexus_GS_450h_F_Sport_Sedan_1_bus : Subsystem  Tag=actuator/StatePort  Priority=0  LoadFcn=load('PreScanStateActuatorData.mat')  mask(PreScan Sink Block: State){}
      mask help: The Actor State contains a vector signal of size (9x1), containing the following signals: - Position (x,y,z) [m] - Velocity (vx,vy,vz) [m/s] - Angles (Roll, Pitch, Yaw) [rad] The Actor state is defined in the global axis system. The state is superponed on the Initial position defined in the GUI. For more information, please click Help.
      settings: OpenFcn=open_system([gcb '/Actuator'],'mask')
      mask Help: eval('openHelp(222)')
      mask Display: image(imread('State.png'))
  STATE_Lexus_LS_600h_F_Sport_1_bus : Subsystem  Tag=actuator/StatePort  Priority=0  LoadFcn=load('PreScanStateActuatorData.mat')  mask(PreScan Sink Block: State){}
      mask help: The Actor State contains a vector signal of size (9x1), containing the following signals: - Position (x,y,z) [m] - Velocity (vx,vy,vz) [m/s] - Angles (Roll, Pitch, Yaw) [rad] The Actor state is defined in the global axis system. The state is superponed on the Initial position defined in the GUI. For more information, please click Help.
      settings: OpenFcn=open_system([gcb '/Actuator'],'mask')
      mask Help: eval('openHelp(222)')
      mask Display: image(imread('State.png'))
  STATE_Male_200_1_bus : Subsystem  Tag=actuator/StatePort  Priority=0  LoadFcn=load('PreScanStateActuatorData.mat')  mask(PreScan Sink Block: State){}
      mask help: The Actor State contains a vector signal of size (9x1), containing the following signals: - Position (x,y,z) [m] - Velocity (vx,vy,vz) [m/s] - Angles (Roll, Pitch, Yaw) [rad] The Actor state is defined in the global axis system. The state is superponed on the Initial position defined in the GUI. For more information, please click Help.
      settings: OpenFcn=open_system([gcb '/Actuator'],'mask')
      mask Help: eval('openHelp(222)')
      mask Display: image(imread('State.png'))
  STATE_Male_African_1_bus : Subsystem  Tag=actuator/StatePort  Priority=0  LoadFcn=load('PreScanStateActuatorData.mat')  mask(PreScan Sink Block: State){}
      mask help: The Actor State contains a vector signal of size (9x1), containing the following signals: - Position (x,y,z) [m] - Velocity (vx,vy,vz) [m/s] - Angles (Roll, Pitch, Yaw) [rad] The Actor state is defined in the global axis system. The state is superponed on the Initial position defined in the GUI. For more information, please click Help.
      settings: OpenFcn=open_system([gcb '/Actuator'],'mask')
      mask Help: eval('openHelp(222)')
      mask Display: image(imread('State.png'))
  STATE_Male_CyclingCyclist_10_bus : Subsystem  Tag=actuator/StatePort  Priority=0  LoadFcn=load('PreScanStateActuatorData.mat')  mask(PreScan Sink Block: State){}
      mask help: The Actor State contains a vector signal of size (9x1), containing the following signals: - Position (x,y,z) [m] - Velocity (vx,vy,vz) [m/s] - Angles (Roll, Pitch, Yaw) [rad] The Actor state is defined in the global axis system. The state is superponed on the Initial position defined in the GUI. For more information, please click Help.
      settings: OpenFcn=open_system([gcb '/Actuator'],'mask')
      mask Help: eval('openHelp(222)')
      mask Display: image(imread('State.png'))
  STATE_Male_CyclingCyclist_1_bus : Subsystem  Tag=actuator/StatePort  Priority=0  LoadFcn=load('PreScanStateActuatorData.mat')  mask(PreScan Sink Block: State){}
      mask help: The Actor State contains a vector signal of size (9x1), containing the following signals: - Position (x,y,z) [m] - Velocity (vx,vy,vz) [m/s] - Angles (Roll, Pitch, Yaw) [rad] The Actor state is defined in the global axis system. The state is superponed on the Initial position defined in the GUI. For more information, please click Help.
      settings: OpenFcn=open_system([gcb '/Actuator'],'mask')
      mask Help: eval('openHelp(222)')
      mask Display: image(imread('State.png'))
  STATE_Male_CyclingCyclist_2_bus : Subsystem  Tag=actuator/StatePort  Priority=0  LoadFcn=load('PreScanStateActuatorData.mat')  mask(PreScan Sink Block: State){}
      mask help: The Actor State contains a vector signal of size (9x1), containing the following signals: - Position (x,y,z) [m] - Velocity (vx,vy,vz) [m/s] - Angles (Roll, Pitch, Yaw) [rad] The Actor state is defined in the global axis system. The state is superponed on the Initial position defined in the GUI. For more information, please click Help.
      settings: OpenFcn=open_system([gcb '/Actuator'],'mask')
      mask Help: eval('openHelp(222)')
      mask Display: image(imread('State.png'))
  STATE_Male_CyclingCyclist_3_bus : Subsystem  Tag=actuator/StatePort  Priority=0  LoadFcn=load('PreScanStateActuatorData.mat')  mask(PreScan Sink Block: State){}
      mask help: The Actor State contains a vector signal of size (9x1), containing the following signals: - Position (x,y,z) [m] - Velocity (vx,vy,vz) [m/s] - Angles (Roll, Pitch, Yaw) [rad] The Actor state is defined in the global axis system. The state is superponed on the Initial position defined in the GUI. For more information, please click Help.
      settings: OpenFcn=open_system([gcb '/Actuator'],'mask')
      mask Help: eval('openHelp(222)')
      mask Display: image(imread('State.png'))
  STATE_Male_CyclingCyclist_4_bus : Subsystem  Tag=actuator/StatePort  Priority=0  LoadFcn=load('PreScanStateActuatorData.mat')  mask(PreScan Sink Block: State){}
      mask help: The Actor State contains a vector signal of size (9x1), containing the following signals: - Position (x,y,z) [m] - Velocity (vx,vy,vz) [m/s] - Angles (Roll, Pitch, Yaw) [rad] The Actor state is defined in the global axis system. The state is superponed on the Initial position defined in the GUI. For more information, please click Help.
      settings: OpenFcn=open_system([gcb '/Actuator'],'mask')
      mask Help: eval('openHelp(222)')
      mask Display: image(imread('State.png'))
  STATE_Male_CyclingCyclist_5_bus : Subsystem  Tag=actuator/StatePort  Priority=0  LoadFcn=load('PreScanStateActuatorData.mat')  mask(PreScan Sink Block: State){}
      mask help: The Actor State contains a vector signal of size (9x1), containing the following signals: - Position (x,y,z) [m] - Velocity (vx,vy,vz) [m/s] - Angles (Roll, Pitch, Yaw) [rad] The Actor state is defined in the global axis system. The state is superponed on the Initial position defined in the GUI. For more information, please click Help.
      settings: OpenFcn=open_system([gcb '/Actuator'],'mask')
      mask Help: eval('openHelp(222)')
      mask Display: image(imread('State.png'))
  STATE_Male_CyclingCyclist_6_bus : Subsystem  Tag=actuator/StatePort  Priority=0  LoadFcn=load('PreScanStateActuatorData.mat')  mask(PreScan Sink Block: State){}
      mask help: The Actor State contains a vector signal of size (9x1), containing the following signals: - Position (x,y,z) [m] - Velocity (vx,vy,vz) [m/s] - Angles (Roll, Pitch, Yaw) [rad] The Actor state is defined in the global axis system. The state is superponed on the Initial position defined in the GUI. For more information, please click Help.
      settings: OpenFcn=open_system([gcb '/Actuator'],'mask')
      mask Help: eval('openHelp(222)')
      mask Display: image(imread('State.png'))
  STATE_Male_CyclingCyclist_7_bus : Subsystem  Tag=actuator/StatePort  Priority=0  LoadFcn=load('PreScanStateActuatorData.mat')  mask(PreScan Sink Block: State){}
      mask help: The Actor State contains a vector signal of size (9x1), containing the following signals: - Position (x,y,z) [m] - Velocity (vx,vy,vz) [m/s] - Angles (Roll, Pitch, Yaw) [rad] The Actor state is defined in the global axis system. The state is superponed on the Initial position defined in the GUI. For more information, please click Help.
      settings: OpenFcn=open_system([gcb '/Actuator'],'mask')
      mask Help: eval('openHelp(222)')
      mask Display: image(imread('State.png'))
  STATE_Male_CyclingCyclist_8_bus : Subsystem  Tag=actuator/StatePort  Priority=0  LoadFcn=load('PreScanStateActuatorData.mat')  mask(PreScan Sink Block: State){}
      mask help: The Actor State contains a vector signal of size (9x1), containing the following signals: - Position (x,y,z) [m] - Velocity (vx,vy,vz) [m/s] - Angles (Roll, Pitch, Yaw) [rad] The Actor state is defined in the global axis system. The state is superponed on the Initial position defined in the GUI. For more information, please click Help.
      settings: OpenFcn=open_system([gcb '/Actuator'],'mask')
      mask Help: eval('openHelp(222)')
      mask Display: image(imread('State.png'))
  STATE_Male_CyclingCyclist_9_bus : Subsystem  Tag=actuator/StatePort  Priority=0  LoadFcn=load('PreScanStateActuatorData.mat')  mask(PreScan Sink Block: State){}
      mask help: The Actor State contains a vector signal of size (9x1), containing the following signals: - Position (x,y,z) [m] - Velocity (vx,vy,vz) [m/s] - Angles (Roll, Pitch, Yaw) [rad] The Actor state is defined in the global axis system. The state is superponed on the Initial position defined in the GUI. For more information, please click Help.
      settings: OpenFcn=open_system([gcb '/Actuator'],'mask')
      mask Help: eval('openHelp(222)')
      mask Display: image(imread('State.png'))
  STATE_Male_LargeShoulderSuitcase_1_bus : Subsystem  Tag=actuator/StatePort  Priority=0  LoadFcn=load('PreScanStateActuatorData.mat')  mask(PreScan Sink Block: State){}
      mask help: The Actor State contains a vector signal of size (9x1), containing the following signals: - Position (x,y,z) [m] - Velocity (vx,vy,vz) [m/s] - Angles (Roll, Pitch, Yaw) [rad] The Actor state is defined in the global axis system. The state is superponed on the Initial position defined in the GUI. For more information, please click Help.
      settings: OpenFcn=open_system([gcb '/Actuator'],'mask')
      mask Help: eval('openHelp(222)')
      mask Display: image(imread('State.png'))
  STATE_Male_Old_White_WithStick_1_bus : Subsystem  Tag=actuator/StatePort  Priority=0  LoadFcn=load('PreScanStateActuatorData.mat')  mask(PreScan Sink Block: State){}
      mask help: The Actor State contains a vector signal of size (9x1), containing the following signals: - Position (x,y,z) [m] - Velocity (vx,vy,vz) [m/s] - Angles (Roll, Pitch, Yaw) [rad] The Actor state is defined in the global axis system. The state is superponed on the Initial position defined in the GUI. For more information, please click Help.
      settings: OpenFcn=open_system([gcb '/Actuator'],'mask')
      mask Help: eval('openHelp(222)')
      mask Display: image(imread('State.png'))
  STATE_Male_Old_White_WithWalkerWithWheels_1_bus : Subsystem  Tag=actuator/StatePort  Priority=0  LoadFcn=load('PreScanStateActuatorData.mat')  mask(PreScan Sink Block: State){}
      mask help: The Actor State contains a vector signal of size (9x1), containing the following signals: - Position (x,y,z) [m] - Velocity (vx,vy,vz) [m/s] - Angles (Roll, Pitch, Yaw) [rad] The Actor state is defined in the global axis system. The state is superponed on the Initial position defined in the GUI. For more information, please click Help.
      settings: OpenFcn=open_system([gcb '/Actuator'],'mask')
      mask Help: eval('openHelp(222)')
      mask Display: image(imread('State.png'))
  STATE_Male_Old_White_WithWalker_1_bus : Subsystem  Tag=actuator/StatePort  Priority=0  LoadFcn=load('PreScanStateActuatorData.mat')  mask(PreScan Sink Block: State){}
      mask help: The Actor State contains a vector signal of size (9x1), containing the following signals: - Position (x,y,z) [m] - Velocity (vx,vy,vz) [m/s] - Angles (Roll, Pitch, Yaw) [rad] The Actor state is defined in the global axis system. The state is superponed on the Initial position defined in the GUI. For more information, please click Help.
      settings: OpenFcn=open_system([gcb '/Actuator'],'mask')
      mask Help: eval('openHelp(222)')
      mask Display: image(imread('State.png'))
  STATE_Male_Overweight_1_bus : Subsystem  Tag=actuator/StatePort  Priority=0  LoadFcn=load('PreScanStateActuatorData.mat')  mask(PreScan Sink Block: State){}
      mask help: The Actor State contains a vector signal of size (9x1), containing the following signals: - Position (x,y,z) [m] - Velocity (vx,vy,vz) [m/s] - Angles (Roll, Pitch, Yaw) [rad] The Actor state is defined in the global axis system. The state is superponed on the Initial position defined in the GUI. For more information, please click Help.
      settings: OpenFcn=open_system([gcb '/Actuator'],'mask')
      mask Help: eval('openHelp(222)')
      mask Display: image(imread('State.png'))
  STATE_Male_ShoppingBag_1_bus : Subsystem  Tag=actuator/StatePort  Priority=0  LoadFcn=load('PreScanStateActuatorData.mat')  mask(PreScan Sink Block: State){}
      mask help: The Actor State contains a vector signal of size (9x1), containing the following signals: - Position (x,y,z) [m] - Velocity (vx,vy,vz) [m/s] - Angles (Roll, Pitch, Yaw) [rad] The Actor state is defined in the global axis system. The state is superponed on the Initial position defined in the GUI. For more information, please click Help.
      settings: OpenFcn=open_system([gcb '/Actuator'],'mask')
      mask Help: eval('openHelp(222)')
      mask Display: image(imread('State.png'))
  STATE_Male_wBackpack_1_bus : Subsystem  Tag=actuator/StatePort  Priority=0  LoadFcn=load('PreScanStateActuatorData.mat')  mask(PreScan Sink Block: State){}
      mask help: The Actor State contains a vector signal of size (9x1), containing the following signals: - Position (x,y,z) [m] - Velocity (vx,vy,vz) [m/s] - Angles (Roll, Pitch, Yaw) [rad] The Actor state is defined in the global axis system. The state is superponed on the Initial position defined in the GUI. For more information, please click Help.
      settings: OpenFcn=open_system([gcb '/Actuator'],'mask')
      mask Help: eval('openHelp(222)')
      mask Display: image(imread('State.png'))
  STATE_Male_wLargeBackpack_1_bus : Subsystem  Tag=actuator/StatePort  Priority=0  LoadFcn=load('PreScanStateActuatorData.mat')  mask(PreScan Sink Block: State){}
      mask help: The Actor State contains a vector signal of size (9x1), containing the following signals: - Position (x,y,z) [m] - Velocity (vx,vy,vz) [m/s] - Angles (Roll, Pitch, Yaw) [rad] The Actor state is defined in the global axis system. The state is superponed on the Initial position defined in the GUI. For more information, please click Help.
      settings: OpenFcn=open_system([gcb '/Actuator'],'mask')
      mask Help: eval('openHelp(222)')
      mask Display: image(imread('State.png'))
  STATE_Male_wLongCoat_1_bus : Subsystem  Tag=actuator/StatePort  Priority=0  LoadFcn=load('PreScanStateActuatorData.mat')  mask(PreScan Sink Block: State){}
      mask help: The Actor State contains a vector signal of size (9x1), containing the following signals: - Position (x,y,z) [m] - Velocity (vx,vy,vz) [m/s] - Angles (Roll, Pitch, Yaw) [rad] The Actor state is defined in the global axis system. The state is superponed on the Initial position defined in the GUI. For more information, please click Help.
      settings: OpenFcn=open_system([gcb '/Actuator'],'mask')
      mask Help: eval('openHelp(222)')
      mask Display: image(imread('State.png'))
  STATE_Male_wSuit_1_bus : Subsystem  Tag=actuator/StatePort  Priority=0  LoadFcn=load('PreScanStateActuatorData.mat')  mask(PreScan Sink Block: State){}
      mask help: The Actor State contains a vector signal of size (9x1), containing the following signals: - Position (x,y,z) [m] - Velocity (vx,vy,vz) [m/s] - Angles (Roll, Pitch, Yaw) [rad] The Actor state is defined in the global axis system. The state is superponed on the Initial position defined in the GUI. For more information, please click Help.
      settings: OpenFcn=open_system([gcb '/Actuator'],'mask')
      mask Help: eval('openHelp(222)')
      mask Display: image(imread('State.png'))
  STATE_Man_250_1_bus : Subsystem  Tag=actuator/StatePort  Priority=0  LoadFcn=load('PreScanStateActuatorData.mat')  mask(PreScan Sink Block: State){}
      mask help: The Actor State contains a vector signal of size (9x1), containing the following signals: - Position (x,y,z) [m] - Velocity (vx,vy,vz) [m/s] - Angles (Roll, Pitch, Yaw) [rad] The Actor state is defined in the global axis system. The state is superponed on the Initial position defined in the GUI. For more information, please click Help.
      settings: OpenFcn=open_system([gcb '/Actuator'],'mask')
      mask Help: eval('openHelp(222)')
      mask Display: image(imread('State.png'))
  STATE_Mazda_RX8_Coupe_1_bus : Subsystem  Tag=actuator/StatePort  Priority=0  LoadFcn=load('PreScanStateActuatorData.mat')  mask(PreScan Sink Block: State){}
      mask help: The Actor State contains a vector signal of size (9x1), containing the following signals: - Position (x,y,z) [m] - Velocity (vx,vy,vz) [m/s] - Angles (Roll, Pitch, Yaw) [rad] The Actor state is defined in the global axis system. The state is superponed on the Initial position defined in the GUI. For more information, please click Help.
      settings: OpenFcn=open_system([gcb '/Actuator'],'mask')
      mask Help: eval('openHelp(222)')
      mask Display: image(imread('State.png'))
  STATE_Roewe_550_S_Sedan_1_bus : Subsystem  Tag=actuator/StatePort  Priority=0  LoadFcn=load('PreScanStateActuatorData.mat')  mask(PreScan Sink Block: State){}
      mask help: The Actor State contains a vector signal of size (9x1), containing the following signals: - Position (x,y,z) [m] - Velocity (vx,vy,vz) [m/s] - Angles (Roll, Pitch, Yaw) [rad] The Actor state is defined in the global axis system. The state is superponed on the Initial position defined in the GUI. For more information, please click Help.
      settings: OpenFcn=open_system([gcb '/Actuator'],'mask')
      mask Help: eval('openHelp(222)')
      mask Display: image(imread('State.png'))
  STATE_Sports_Bike_wDriver_1_bus : Subsystem  Tag=actuator/StatePort  Priority=0  LoadFcn=load('PreScanStateActuatorData.mat')  mask(PreScan Sink Block: State){}
      mask help: The Actor State contains a vector signal of size (9x1), containing the following signals: - Position (x,y,z) [m] - Velocity (vx,vy,vz) [m/s] - Angles (Roll, Pitch, Yaw) [rad] The Actor state is defined in the global axis system. The state is superponed on the Initial position defined in the GUI. For more information, please click Help.
      settings: OpenFcn=open_system([gcb '/Actuator'],'mask')
      mask Help: eval('openHelp(222)')
      mask Display: image(imread('State.png'))
  STATE_Sports_Bike_wDriver_2_bus : Subsystem  Tag=actuator/StatePort  Priority=0  LoadFcn=load('PreScanStateActuatorData.mat')  mask(PreScan Sink Block: State){}
      mask help: The Actor State contains a vector signal of size (9x1), containing the following signals: - Position (x,y,z) [m] - Velocity (vx,vy,vz) [m/s] - Angles (Roll, Pitch, Yaw) [rad] The Actor state is defined in the global axis system. The state is superponed on the Initial position defined in the GUI. For more information, please click Help.
      settings: OpenFcn=open_system([gcb '/Actuator'],'mask')
      mask Help: eval('openHelp(222)')
      mask Display: image(imread('State.png'))
  STATE_Sports_Bike_wDriver_3_bus : Subsystem  Tag=actuator/StatePort  Priority=0  LoadFcn=load('PreScanStateActuatorData.mat')  mask(PreScan Sink Block: State){}
      mask help: The Actor State contains a vector signal of size (9x1), containing the following signals: - Position (x,y,z) [m] - Velocity (vx,vy,vz) [m/s] - Angles (Roll, Pitch, Yaw) [rad] The Actor state is defined in the global axis system. The state is superponed on the Initial position defined in the GUI. For more information, please click Help.
      settings: OpenFcn=open_system([gcb '/Actuator'],'mask')
      mask Help: eval('openHelp(222)')
      mask Display: image(imread('State.png'))
  STATE_Tesla_Model_3_1_bus : Subsystem  Tag=actuator/StatePort  Priority=0  LoadFcn=load('PreScanStateActuatorData.mat')  mask(PreScan Sink Block: State){}
      mask help: The Actor State contains a vector signal of size (9x1), containing the following signals: - Position (x,y,z) [m] - Velocity (vx,vy,vz) [m/s] - Angles (Roll, Pitch, Yaw) [rad] The Actor state is defined in the global axis system. The state is superponed on the Initial position defined in the GUI. For more information, please click Help.
      settings: OpenFcn=open_system([gcb '/Actuator'],'mask')
      mask Help: eval('openHelp(222)')
      mask Display: image(imread('State.png'))
  STATE_Toyota_Previa_MPV_1_bus : Subsystem  Tag=actuator/StatePort  Priority=0  LoadFcn=load('PreScanStateActuatorData.mat')  mask(PreScan Sink Block: State){}
      mask help: The Actor State contains a vector signal of size (9x1), containing the following signals: - Position (x,y,z) [m] - Velocity (vx,vy,vz) [m/s] - Angles (Roll, Pitch, Yaw) [rad] The Actor state is defined in the global axis system. The state is superponed on the Initial position defined in the GUI. For more information, please click Help.
      settings: OpenFcn=open_system([gcb '/Actuator'],'mask')
      mask Help: eval('openHelp(222)')
      mask Display: image(imread('State.png'))
  STATE_Toyota_Prius_Sedan_1_bus : Subsystem  Tag=actuator/StatePort  Priority=0  LoadFcn=load('PreScanStateActuatorData.mat')  mask(PreScan Sink Block: State){}
      mask help: The Actor State contains a vector signal of size (9x1), containing the following signals: - Position (x,y,z) [m] - Velocity (vx,vy,vz) [m/s] - Angles (Roll, Pitch, Yaw) [rad] The Actor state is defined in the global axis system. The state is superponed on the Initial position defined in the GUI. For more information, please click Help.
      settings: OpenFcn=open_system([gcb '/Actuator'],'mask')
      mask Help: eval('openHelp(222)')
      mask Display: image(imread('State.png'))
  STATE_Toyota_Yaris_Hatchback_1_bus : Subsystem  Tag=actuator/StatePort  Priority=0  LoadFcn=load('PreScanStateActuatorData.mat')  mask(PreScan Sink Block: State){}
      mask help: The Actor State contains a vector signal of size (9x1), containing the following signals: - Position (x,y,z) [m] - Velocity (vx,vy,vz) [m/s] - Angles (Roll, Pitch, Yaw) [rad] The Actor state is defined in the global axis system. The state is superponed on the Initial position defined in the GUI. For more information, please click Help.
      settings: OpenFcn=open_system([gcb '/Actuator'],'mask')
      mask Help: eval('openHelp(222)')
      mask Display: image(imread('State.png'))
  STATE_Toyota_Yaris_Hatchback_2_bus : Subsystem  Tag=actuator/StatePort  Priority=0  LoadFcn=load('PreScanStateActuatorData.mat')  mask(PreScan Sink Block: State){}
      mask help: The Actor State contains a vector signal of size (9x1), containing the following signals: - Position (x,y,z) [m] - Velocity (vx,vy,vz) [m/s] - Angles (Roll, Pitch, Yaw) [rad] The Actor state is defined in the global axis system. The state is superponed on the Initial position defined in the GUI. For more information, please click Help.
      settings: OpenFcn=open_system([gcb '/Actuator'],'mask')
      mask Help: eval('openHelp(222)')
      mask Display: image(imread('State.png'))
  STATE_Volvo_XC60_1_bus : Subsystem  Tag=actuator/StatePort  Priority=0  LoadFcn=load('PreScanStateActuatorData.mat')  mask(PreScan Sink Block: State){}
      mask help: The Actor State contains a vector signal of size (9x1), containing the following signals: - Position (x,y,z) [m] - Velocity (vx,vy,vz) [m/s] - Angles (Roll, Pitch, Yaw) [rad] The Actor state is defined in the global axis system. The state is superponed on the Initial position defined in the GUI. For more information, please click Help.
      settings: OpenFcn=open_system([gcb '/Actuator'],'mask')
      mask Help: eval('openHelp(222)')
      mask Display: image(imread('State.png'))
  STATE_Wuling_Hongguang_1_bus : Subsystem  Tag=actuator/StatePort  Priority=0  LoadFcn=load('PreScanStateActuatorData.mat')  mask(PreScan Sink Block: State){}
      mask help: The Actor State contains a vector signal of size (9x1), containing the following signals: - Position (x,y,z) [m] - Velocity (vx,vy,vz) [m/s] - Angles (Roll, Pitch, Yaw) [rad] The Actor state is defined in the global axis system. The state is superponed on the Initial position defined in the GUI. For more information, please click Help.
      settings: OpenFcn=open_system([gcb '/Actuator'],'mask')
      mask Help: eval('openHelp(222)')
      mask Display: image(imread('State.png'))
  ScenarioEngine : Subsystem  Tag=PreScanOpenScenarioBlock  Priority=10  LoadFcn=load PrescanSynchronizeData  mask(PreScan Simulation Core Block){TimeStep=1/20}
      mask prompts: TimeStep "Timestep [s]"
      mask help: Please do not remove this block from the PreScan compilation sheet, as it contains essential configuration parameters for a PreScan simulation.
      settings: DeleteFcn=PreScanBlockDeleteFcn;
      mask Display: image(imread('prescanlogo.ico'))
  Sports_Bike_wDriver_1 : Subsystem  Tag=WorldObjectSubSystem  InitFcn=UniqueId = '29036';
      mask init:
      | modelPath = GenericModelHelper.getGenericModelFilePath('ModelDepo','Vehicles\Sports_Bike_wDriver\Sports_Bike_wDriver.pgmb','b225a47241fa9a095f8ef185f38a78e4');imagePath = GenericModelHelper.getCompilationPicture(modelPath, 'Sports_Bike_wDriver.png');
      mask Display: image(imread(imagePath));color('white');text(0, 0, ' ID=120\n')
  Sports_Bike_wDriver_2 : Subsystem  Tag=WorldObjectSubSystem  InitFcn=UniqueId = '29106';
      mask init: same as W01_Base_Map_cs/Sports_Bike_wDriver_1
      mask Display: image(imread(imagePath));color('white');text(0, 0, ' ID=155\n')
  Sports_Bike_wDriver_3 : Subsystem  Tag=WorldObjectSubSystem  InitFcn=UniqueId = '29107';
      mask init: same as W01_Base_Map_cs/Sports_Bike_wDriver_1
      mask Display: image(imread(imagePath));color('white');text(0, 0, ' ID=156\n')
  Subsystem : Subsystem
  Synchronizer : Subsystem  Tag=PreScanSynchronizer  Priority=20  LoadFcn=load PrescanSynchronizeData  mask(PreScan Simulation Core Block){TimeStep=1/20}
      mask prompts: TimeStep "Timestep [s]"
      mask help: Please do not remove this block from the PreScan compilation sheet, as it contains essential configuration parameters for a PreScan simulation.
      settings: DeleteFcn=PreScanBlockDeleteFcn;
      mask Display: image(imread('prescanlogo.ico'))
  Tesla_Model_3_1 : Subsystem  Tag=WorldObjectSubSystem  InitFcn=UniqueId = '29037';
      mask init:
      | modelPath = GenericModelHelper.getGenericModelFilePath('ModelDepo','Vehicles\TeslaModel3\TeslaModel3.pgmb','098e3ab7f5fc6e82510eadc212c66ee7');imagePath = GenericModelHelper.getCompilationPicture(modelPath, 'TeslaModel3.png');
      mask Display: image(imread(imagePath));color('white');text(0, 0, ' ID=121\n')
  Toyota_Previa_MPV_1 : Subsystem  Tag=WorldObjectSubSystem  InitFcn=UniqueId = '29072';
      mask init:
      | modelPath = GenericModelHelper.getGenericModelFilePath('ModelDepo','Vehicles\Toyota_Previa\Toyota_Previa.pgmb','93e58f95175b34f6ce91a88cdfe55b40');imagePath = GenericModelHelper.getCompilationPicture(modelPath, 'Toyota_Previa_HighPoly.png');
      mask Display: image(imread(imagePath));color('white');text(0, 0, ' ID=148\n')
  Toyota_Prius_Sedan_1 : Subsystem  Tag=WorldObjectSubSystem  InitFcn=UniqueId = '29073';
      mask init:
      | modelPath = GenericModelHelper.getGenericModelFilePath('ModelDepo','Vehicles\Toyota_Prius\Toyota_Prius.pgmb','756f4989efba73a9bc798074a2dfdeb4');imagePath = GenericModelHelper.getCompilationPicture(modelPath, 'Toyota_Prius_HighPoly.png');
      mask Display: image(imread(imagePath));color('white');text(0, 0, ' ID=149\n')
  Toyota_Yaris_Hatchback_1 : Subsystem  Tag=WorldObjectSubSystem  InitFcn=UniqueId = '29074';
      mask init:
      | modelPath = GenericModelHelper.getGenericModelFilePath('ModelDepo','Vehicles\Toyota_Yaris\Toyota_Yaris.pgmb','3ea2b9be97d70b5ca322b210574befd9');imagePath = GenericModelHelper.getCompilationPicture(modelPath, 'Toyota_Yaris_HighPoly.png');
      mask Display: image(imread(imagePath));color('white');text(0, 0, ' ID=150\n')
  Toyota_Yaris_Hatchback_2 : Subsystem  Tag=WorldObjectSubSystem  InitFcn=UniqueId = '29076';
      mask init: same as W01_Base_Map_cs/Toyota_Yaris_Hatchback_1
      mask Display: image(imread(imagePath));color('white');text(0, 0, ' ID=152\n')
  TrafficLightRoadSideNL_1 : Subsystem  Tag=WorldObjectSubSystem  InitFcn=UniqueId = '646';
      mask init:
      | modelPath = GenericModelHelper.getGenericModelFilePath('ModelDepo','AnimatedElements\TrafficLight_NL\Roadside\Roadside_NL.pgmb','2000fba5e1a6d0fba32e88146243c3cb');imagePath = GenericModelHelper.getCompilationPicture(modelPath, 'Roadside_NL.png');
      mask Display: image(imread(imagePath));color('white');text(0, 0, ' ID=76\n')
  TrafficLightRoadSideNL_1_Green : Subsystem  Tag=actuator/Green  Priority=0  LoadFcn=load('PreScanVisuLightActuatorData');load('PrescanRPYData');load('PrescanXYZData');load('PreScanRGBData')  mask(PreScan Sink Block: VisuActiveLight){}
      mask help: The VisuActiveLight block provides a way for detailed animation of Light Sources, such as the indicator, brake, fog and main lights of a vehicle, or a light post. For more information, please click Help.
      settings: OpenFcn=open_system([gcb '/Actuator'],'mask')
      mask Help: eval('openHelp(209)')
      mask Display: image(imread('HeadLight.png'))
  TrafficLightRoadSideNL_1_Orange : Subsystem  Tag=actuator/Orange  Priority=0  LoadFcn=load('PreScanVisuLightActuatorData');load('PrescanRPYData');load('PrescanXYZData');load('PreScanRGBData')  mask(PreScan Sink Block: VisuActiveLight){}
      mask help: The VisuActiveLight block provides a way for detailed animation of Light Sources, such as the indicator, brake, fog and main lights of a vehicle, or a light post. For more information, please click Help.
      settings: OpenFcn=open_system([gcb '/Actuator'],'mask')
      mask Help: eval('openHelp(209)')
      mask Display: image(imread('HeadLight.png'))
  TrafficLightRoadSideNL_1_Red : Subsystem  Tag=actuator/Red  Priority=0  LoadFcn=load('PreScanVisuLightActuatorData');load('PrescanRPYData');load('PrescanXYZData');load('PreScanRGBData')  mask(PreScan Sink Block: VisuActiveLight){}
      mask help: The VisuActiveLight block provides a way for detailed animation of Light Sources, such as the indicator, brake, fog and main lights of a vehicle, or a light post. For more information, please click Help.
      settings: OpenFcn=open_system([gcb '/Actuator'],'mask')
      mask Help: eval('openHelp(209)')
      mask Display: image(imread('HeadLight.png'))
  TrafficLightRoadSideNL_2 : Subsystem  Tag=WorldObjectSubSystem  InitFcn=UniqueId = '647';
      mask init: same as W01_Base_Map_cs/TrafficLightRoadSideNL_1
      mask Display: image(imread(imagePath));color('white');text(0, 0, ' ID=77\n')
  TrafficLightRoadSideNL_2_Green : Subsystem  Tag=actuator/Green  Priority=0  LoadFcn=load('PreScanVisuLightActuatorData');load('PrescanRPYData');load('PrescanXYZData');load('PreScanRGBData')  mask(PreScan Sink Block: VisuActiveLight){}
      mask help: The VisuActiveLight block provides a way for detailed animation of Light Sources, such as the indicator, brake, fog and main lights of a vehicle, or a light post. For more information, please click Help.
      settings: OpenFcn=open_system([gcb '/Actuator'],'mask')
      mask Help: eval('openHelp(209)')
      mask Display: image(imread('HeadLight.png'))
  TrafficLightRoadSideNL_2_Orange : Subsystem  Tag=actuator/Orange  Priority=0  LoadFcn=load('PreScanVisuLightActuatorData');load('PrescanRPYData');load('PrescanXYZData');load('PreScanRGBData')  mask(PreScan Sink Block: VisuActiveLight){}
      mask help: The VisuActiveLight block provides a way for detailed animation of Light Sources, such as the indicator, brake, fog and main lights of a vehicle, or a light post. For more information, please click Help.
      settings: OpenFcn=open_system([gcb '/Actuator'],'mask')
      mask Help: eval('openHelp(209)')
      mask Display: image(imread('HeadLight.png'))
  TrafficLightRoadSideNL_2_Red : Subsystem  Tag=actuator/Red  Priority=0  LoadFcn=load('PreScanVisuLightActuatorData');load('PrescanRPYData');load('PrescanXYZData');load('PreScanRGBData')  mask(PreScan Sink Block: VisuActiveLight){}
      mask help: The VisuActiveLight block provides a way for detailed animation of Light Sources, such as the indicator, brake, fog and main lights of a vehicle, or a light post. For more information, please click Help.
      settings: OpenFcn=open_system([gcb '/Actuator'],'mask')
      mask Help: eval('openHelp(209)')
      mask Display: image(imread('HeadLight.png'))
  TrafficLightRoadSideNL_3 : Subsystem  Tag=WorldObjectSubSystem  InitFcn=UniqueId = '649';
      mask init: same as W01_Base_Map_cs/TrafficLightRoadSideNL_1
      mask Display: image(imread(imagePath));color('white');text(0, 0, ' ID=78\n')
  TrafficLightRoadSideNL_3_Green : Subsystem  Tag=actuator/Green  Priority=0  LoadFcn=load('PreScanVisuLightActuatorData');load('PrescanRPYData');load('PrescanXYZData');load('PreScanRGBData')  mask(PreScan Sink Block: VisuActiveLight){}
      mask help: The VisuActiveLight block provides a way for detailed animation of Light Sources, such as the indicator, brake, fog and main lights of a vehicle, or a light post. For more information, please click Help.
      settings: OpenFcn=open_system([gcb '/Actuator'],'mask')
      mask Help: eval('openHelp(209)')
      mask Display: image(imread('HeadLight.png'))
  TrafficLightRoadSideNL_3_Orange : Subsystem  Tag=actuator/Orange  Priority=0  LoadFcn=load('PreScanVisuLightActuatorData');load('PrescanRPYData');load('PrescanXYZData');load('PreScanRGBData')  mask(PreScan Sink Block: VisuActiveLight){}
      mask help: The VisuActiveLight block provides a way for detailed animation of Light Sources, such as the indicator, brake, fog and main lights of a vehicle, or a light post. For more information, please click Help.
      settings: OpenFcn=open_system([gcb '/Actuator'],'mask')
      mask Help: eval('openHelp(209)')
      mask Display: image(imread('HeadLight.png'))
  TrafficLightRoadSideNL_3_Red : Subsystem  Tag=actuator/Red  Priority=0  LoadFcn=load('PreScanVisuLightActuatorData');load('PrescanRPYData');load('PrescanXYZData');load('PreScanRGBData')  mask(PreScan Sink Block: VisuActiveLight){}
      mask help: The VisuActiveLight block provides a way for detailed animation of Light Sources, such as the indicator, brake, fog and main lights of a vehicle, or a light post. For more information, please click Help.
      settings: OpenFcn=open_system([gcb '/Actuator'],'mask')
      mask Help: eval('openHelp(209)')
      mask Display: image(imread('HeadLight.png'))
  TrafficLightRoadSideNL_4 : Subsystem  Tag=WorldObjectSubSystem  InitFcn=UniqueId = '650';
      mask init: same as W01_Base_Map_cs/TrafficLightRoadSideNL_1
      mask Display: image(imread(imagePath));color('white');text(0, 0, ' ID=79\n')
  TrafficLightRoadSideNL_4_Green : Subsystem  Tag=actuator/Green  Priority=0  LoadFcn=load('PreScanVisuLightActuatorData');load('PrescanRPYData');load('PrescanXYZData');load('PreScanRGBData')  mask(PreScan Sink Block: VisuActiveLight){}
      mask help: The VisuActiveLight block provides a way for detailed animation of Light Sources, such as the indicator, brake, fog and main lights of a vehicle, or a light post. For more information, please click Help.
      settings: OpenFcn=open_system([gcb '/Actuator'],'mask')
      mask Help: eval('openHelp(209)')
      mask Display: image(imread('HeadLight.png'))
  TrafficLightRoadSideNL_4_Orange : Subsystem  Tag=actuator/Orange  Priority=0  LoadFcn=load('PreScanVisuLightActuatorData');load('PrescanRPYData');load('PrescanXYZData');load('PreScanRGBData')  mask(PreScan Sink Block: VisuActiveLight){}
      mask help: The VisuActiveLight block provides a way for detailed animation of Light Sources, such as the indicator, brake, fog and main lights of a vehicle, or a light post. For more information, please click Help.
      settings: OpenFcn=open_system([gcb '/Actuator'],'mask')
      mask Help: eval('openHelp(209)')
      mask Display: image(imread('HeadLight.png'))
  TrafficLightRoadSideNL_4_Red : Subsystem  Tag=actuator/Red  Priority=0  LoadFcn=load('PreScanVisuLightActuatorData');load('PrescanRPYData');load('PrescanXYZData');load('PreScanRGBData')  mask(PreScan Sink Block: VisuActiveLight){}
      mask help: The VisuActiveLight block provides a way for detailed animation of Light Sources, such as the indicator, brake, fog and main lights of a vehicle, or a light post. For more information, please click Help.
      settings: OpenFcn=open_system([gcb '/Actuator'],'mask')
      mask Help: eval('openHelp(209)')
      mask Display: image(imread('HeadLight.png'))
  TrafficLightRoadSideNL_5 : Subsystem  Tag=WorldObjectSubSystem  InitFcn=UniqueId = '651';
      mask init: same as W01_Base_Map_cs/TrafficLightRoadSideNL_1
      mask Display: image(imread(imagePath));color('white');text(0, 0, ' ID=80\n')
  TrafficLightRoadSideNL_5_Green : Subsystem  Tag=actuator/Green  Priority=0  LoadFcn=load('PreScanVisuLightActuatorData');load('PrescanRPYData');load('PrescanXYZData');load('PreScanRGBData')  mask(PreScan Sink Block: VisuActiveLight){}
      mask help: The VisuActiveLight block provides a way for detailed animation of Light Sources, such as the indicator, brake, fog and main lights of a vehicle, or a light post. For more information, please click Help.
      settings: OpenFcn=open_system([gcb '/Actuator'],'mask')
      mask Help: eval('openHelp(209)')
      mask Display: image(imread('HeadLight.png'))
  TrafficLightRoadSideNL_5_Orange : Subsystem  Tag=actuator/Orange  Priority=0  LoadFcn=load('PreScanVisuLightActuatorData');load('PrescanRPYData');load('PrescanXYZData');load('PreScanRGBData')  mask(PreScan Sink Block: VisuActiveLight){}
      mask help: The VisuActiveLight block provides a way for detailed animation of Light Sources, such as the indicator, brake, fog and main lights of a vehicle, or a light post. For more information, please click Help.
      settings: OpenFcn=open_system([gcb '/Actuator'],'mask')
      mask Help: eval('openHelp(209)')
      mask Display: image(imread('HeadLight.png'))
  TrafficLightRoadSideNL_5_Red : Subsystem  Tag=actuator/Red  Priority=0  LoadFcn=load('PreScanVisuLightActuatorData');load('PrescanRPYData');load('PrescanXYZData');load('PreScanRGBData')  mask(PreScan Sink Block: VisuActiveLight){}
      mask help: The VisuActiveLight block provides a way for detailed animation of Light Sources, such as the indicator, brake, fog and main lights of a vehicle, or a light post. For more information, please click Help.
      settings: OpenFcn=open_system([gcb '/Actuator'],'mask')
      mask Help: eval('openHelp(209)')
      mask Display: image(imread('HeadLight.png'))
  TrafficLightRoadSideNL_6 : Subsystem  Tag=WorldObjectSubSystem  InitFcn=UniqueId = '10446';
      mask init: same as W01_Base_Map_cs/TrafficLightRoadSideNL_1
      mask Display: image(imread(imagePath));color('white');text(0, 0, ' ID=81\n')
  TrafficLightRoadSideNL_6_Green : Subsystem  Tag=actuator/Green  Priority=0  LoadFcn=load('PreScanVisuLightActuatorData');load('PrescanRPYData');load('PrescanXYZData');load('PreScanRGBData')  mask(PreScan Sink Block: VisuActiveLight){}
      mask help: The VisuActiveLight block provides a way for detailed animation of Light Sources, such as the indicator, brake, fog and main lights of a vehicle, or a light post. For more information, please click Help.
      settings: OpenFcn=open_system([gcb '/Actuator'],'mask')
      mask Help: eval('openHelp(209)')
      mask Display: image(imread('HeadLight.png'))
  TrafficLightRoadSideNL_6_Orange : Subsystem  Tag=actuator/Orange  Priority=0  LoadFcn=load('PreScanVisuLightActuatorData');load('PrescanRPYData');load('PrescanXYZData');load('PreScanRGBData')  mask(PreScan Sink Block: VisuActiveLight){}
      mask help: The VisuActiveLight block provides a way for detailed animation of Light Sources, such as the indicator, brake, fog and main lights of a vehicle, or a light post. For more information, please click Help.
      settings: OpenFcn=open_system([gcb '/Actuator'],'mask')
      mask Help: eval('openHelp(209)')
      mask Display: image(imread('HeadLight.png'))
  TrafficLightRoadSideNL_6_Red : Subsystem  Tag=actuator/Red  Priority=0  LoadFcn=load('PreScanVisuLightActuatorData');load('PrescanRPYData');load('PrescanXYZData');load('PreScanRGBData')  mask(PreScan Sink Block: VisuActiveLight){}
      mask help: The VisuActiveLight block provides a way for detailed animation of Light Sources, such as the indicator, brake, fog and main lights of a vehicle, or a light post. For more information, please click Help.
      settings: OpenFcn=open_system([gcb '/Actuator'],'mask')
      mask Help: eval('openHelp(209)')
      mask Display: image(imread('HeadLight.png'))
  TrafficLightRoadSideNL_7 : Subsystem  Tag=WorldObjectSubSystem  InitFcn=UniqueId = '653';
      mask init: same as W01_Base_Map_cs/TrafficLightRoadSideNL_1
      mask Display: image(imread(imagePath));color('white');text(0, 0, ' ID=82\n')
  TrafficLightRoadSideNL_7_Green : Subsystem  Tag=actuator/Green  Priority=0  LoadFcn=load('PreScanVisuLightActuatorData');load('PrescanRPYData');load('PrescanXYZData');load('PreScanRGBData')  mask(PreScan Sink Block: VisuActiveLight){}
      mask help: The VisuActiveLight block provides a way for detailed animation of Light Sources, such as the indicator, brake, fog and main lights of a vehicle, or a light post. For more information, please click Help.
      settings: OpenFcn=open_system([gcb '/Actuator'],'mask')
      mask Help: eval('openHelp(209)')
      mask Display: image(imread('HeadLight.png'))
  TrafficLightRoadSideNL_7_Orange : Subsystem  Tag=actuator/Orange  Priority=0  LoadFcn=load('PreScanVisuLightActuatorData');load('PrescanRPYData');load('PrescanXYZData');load('PreScanRGBData')  mask(PreScan Sink Block: VisuActiveLight){}
      mask help: The VisuActiveLight block provides a way for detailed animation of Light Sources, such as the indicator, brake, fog and main lights of a vehicle, or a light post. For more information, please click Help.
      settings: OpenFcn=open_system([gcb '/Actuator'],'mask')
      mask Help: eval('openHelp(209)')
      mask Display: image(imread('HeadLight.png'))
  TrafficLightRoadSideNL_7_Red : Subsystem  Tag=actuator/Red  Priority=0  LoadFcn=load('PreScanVisuLightActuatorData');load('PrescanRPYData');load('PrescanXYZData');load('PreScanRGBData')  mask(PreScan Sink Block: VisuActiveLight){}
      mask help: The VisuActiveLight block provides a way for detailed animation of Light Sources, such as the indicator, brake, fog and main lights of a vehicle, or a light post. For more information, please click Help.
      settings: OpenFcn=open_system([gcb '/Actuator'],'mask')
      mask Help: eval('openHelp(209)')
      mask Display: image(imread('HeadLight.png'))
  TrafficLightRoadSideNL_8 : Subsystem  Tag=WorldObjectSubSystem  InitFcn=UniqueId = '654';
      mask init: same as W01_Base_Map_cs/TrafficLightRoadSideNL_1
      mask Display: image(imread(imagePath));color('white');text(0, 0, ' ID=83\n')
  TrafficLightRoadSideNL_8_Green : Subsystem  Tag=actuator/Green  Priority=0  LoadFcn=load('PreScanVisuLightActuatorData');load('PrescanRPYData');load('PrescanXYZData');load('PreScanRGBData')  mask(PreScan Sink Block: VisuActiveLight){}
      mask help: The VisuActiveLight block provides a way for detailed animation of Light Sources, such as the indicator, brake, fog and main lights of a vehicle, or a light post. For more information, please click Help.
      settings: OpenFcn=open_system([gcb '/Actuator'],'mask')
      mask Help: eval('openHelp(209)')
      mask Display: image(imread('HeadLight.png'))
  TrafficLightRoadSideNL_8_Orange : Subsystem  Tag=actuator/Orange  Priority=0  LoadFcn=load('PreScanVisuLightActuatorData');load('PrescanRPYData');load('PrescanXYZData');load('PreScanRGBData')  mask(PreScan Sink Block: VisuActiveLight){}
      mask help: The VisuActiveLight block provides a way for detailed animation of Light Sources, such as the indicator, brake, fog and main lights of a vehicle, or a light post. For more information, please click Help.
      settings: OpenFcn=open_system([gcb '/Actuator'],'mask')
      mask Help: eval('openHelp(209)')
      mask Display: image(imread('HeadLight.png'))
  TrafficLightRoadSideNL_8_Red : Subsystem  Tag=actuator/Red  Priority=0  LoadFcn=load('PreScanVisuLightActuatorData');load('PrescanRPYData');load('PrescanXYZData');load('PreScanRGBData')  mask(PreScan Sink Block: VisuActiveLight){}
      mask help: The VisuActiveLight block provides a way for detailed animation of Light Sources, such as the indicator, brake, fog and main lights of a vehicle, or a light post. For more information, please click Help.
      settings: OpenFcn=open_system([gcb '/Actuator'],'mask')
      mask Help: eval('openHelp(209)')
      mask Display: image(imread('HeadLight.png'))
  VISUColorRegion_Bag_Male_LargeShoulderSuitcase_1 : Subsystem  Tag=actuator/ColorRegion  Priority=0  LoadFcn=load('PrescanColorData')  mask(PreScan Sink Block: VisuTextureColor){}
      mask help: The VisuTextureColor block provides a way to adapt the color of a vehicle. For more information, please click Help.
      settings: OpenFcn=open_system([gcb '/Actuator'],'mask')
      mask Help: eval('openHelp(230)')
      mask Display: image(imread('TextureColor.png'))
  VISUColorRegion_Bag_Male_ShoppingBag_1 : Subsystem  Tag=actuator/ColorRegion  Priority=0  LoadFcn=load('PrescanColorData')  mask(PreScan Sink Block: VisuTextureColor){}
      mask help: The VisuTextureColor block provides a way to adapt the color of a vehicle. For more information, please click Help.
      settings: OpenFcn=open_system([gcb '/Actuator'],'mask')
      mask Help: eval('openHelp(230)')
      mask Display: image(imread('TextureColor.png'))
  VISUColorRegion_Bag_Male_wLargeBackpack_1 : Subsystem  Tag=actuator/ColorRegion  Priority=0  LoadFcn=load('PrescanColorData')  mask(PreScan Sink Block: VisuTextureColor){}
      mask help: The VisuTextureColor block provides a way to adapt the color of a vehicle. For more information, please click Help.
      settings: OpenFcn=open_system([gcb '/Actuator'],'mask')
      mask Help: eval('openHelp(230)')
      mask Display: image(imread('TextureColor.png'))
  VISUColorRegion_Coat_Male_wLongCoat_1 : Subsystem  Tag=actuator/ColorRegion  Priority=0  LoadFcn=load('PrescanColorData')  mask(PreScan Sink Block: VisuTextureColor){}
      mask help: The VisuTextureColor block provides a way to adapt the color of a vehicle. For more information, please click Help.
      settings: OpenFcn=open_system([gcb '/Actuator'],'mask')
      mask Help: eval('openHelp(230)')
      mask Display: image(imread('TextureColor.png'))
  VISUColorRegion_Lower_Body_Boy_150_1 : Subsystem  Tag=actuator/ColorRegion  Priority=0  LoadFcn=load('PrescanColorData')  mask(PreScan Sink Block: VisuTextureColor){}
      mask help: The VisuTextureColor block provides a way to adapt the color of a vehicle. For more information, please click Help.
      settings: OpenFcn=open_system([gcb '/Actuator'],'mask')
      mask Help: eval('openHelp(230)')
      mask Display: image(imread('TextureColor.png'))
  VISUColorRegion_Lower_Body_Child_Overweight_1 : Subsystem  Tag=actuator/ColorRegion  Priority=0  LoadFcn=load('PrescanColorData')  mask(PreScan Sink Block: VisuTextureColor){}
      mask help: The VisuTextureColor block provides a way to adapt the color of a vehicle. For more information, please click Help.
      settings: OpenFcn=open_system([gcb '/Actuator'],'mask')
      mask Help: eval('openHelp(230)')
      mask Display: image(imread('TextureColor.png'))
  VISUColorRegion_Lower_Body_Female_Overweight_1 : Subsystem  Tag=actuator/ColorRegion  Priority=0  LoadFcn=load('PrescanColorData')  mask(PreScan Sink Block: VisuTextureColor){}
      mask help: The VisuTextureColor block provides a way to adapt the color of a vehicle. For more information, please click Help.
      settings: OpenFcn=open_system([gcb '/Actuator'],'mask')
      mask Help: eval('openHelp(230)')
      mask Display: image(imread('TextureColor.png'))
  VISUColorRegion_Lower_Body_Female_Regular_1 : Subsystem  Tag=actuator/ColorRegion  Priority=0  LoadFcn=load('PrescanColorData')  mask(PreScan Sink Block: VisuTextureColor){}
      mask help: The VisuTextureColor block provides a way to adapt the color of a vehicle. For more information, please click Help.
      settings: OpenFcn=open_system([gcb '/Actuator'],'mask')
      mask Help: eval('openHelp(230)')
      mask Display: image(imread('TextureColor.png'))
  VISUColorRegion_Lower_Body_Female_wBuggy_1 : Subsystem  Tag=actuator/ColorRegion  Priority=0  LoadFcn=load('PrescanColorData')  mask(PreScan Sink Block: VisuTextureColor){}
      mask help: The VisuTextureColor block provides a way to adapt the color of a vehicle. For more information, please click Help.
      settings: OpenFcn=open_system([gcb '/Actuator'],'mask')
      mask Help: eval('openHelp(230)')
      mask Display: image(imread('TextureColor.png'))
  VISUColorRegion_Lower_Body_Female_wLongCoat_1 : Subsystem  Tag=actuator/ColorRegion  Priority=0  LoadFcn=load('PrescanColorData')  mask(PreScan Sink Block: VisuTextureColor){}
      mask help: The VisuTextureColor block provides a way to adapt the color of a vehicle. For more information, please click Help.
      settings: OpenFcn=open_system([gcb '/Actuator'],'mask')
      mask Help: eval('openHelp(230)')
      mask Display: image(imread('TextureColor.png'))
  VISUColorRegion_Lower_Body_Female_wRaincoat_1 : Subsystem  Tag=actuator/ColorRegion  Priority=0  LoadFcn=load('PrescanColorData')  mask(PreScan Sink Block: VisuTextureColor){}
      mask help: The VisuTextureColor block provides a way to adapt the color of a vehicle. For more information, please click Help.
      settings: OpenFcn=open_system([gcb '/Actuator'],'mask')
      mask Help: eval('openHelp(230)')
      mask Display: image(imread('TextureColor.png'))
  VISUColorRegion_Lower_Body_Male_200_1 : Subsystem  Tag=actuator/ColorRegion  Priority=0  LoadFcn=load('PrescanColorData')  mask(PreScan Sink Block: VisuTextureColor){}
      mask help: The VisuTextureColor block provides a way to adapt the color of a vehicle. For more information, please click Help.
      settings: OpenFcn=open_system([gcb '/Actuator'],'mask')
      mask Help: eval('openHelp(230)')
      mask Display: image(imread('TextureColor.png'))
  VISUColorRegion_Lower_Body_Male_African_1 : Subsystem  Tag=actuator/ColorRegion  Priority=0  LoadFcn=load('PrescanColorData')  mask(PreScan Sink Block: VisuTextureColor){}
      mask help: The VisuTextureColor block provides a way to adapt the color of a vehicle. For more information, please click Help.
      settings: OpenFcn=open_system([gcb '/Actuator'],'mask')
      mask Help: eval('openHelp(230)')
      mask Display: image(imread('TextureColor.png'))
  VISUColorRegion_Lower_Body_Male_LargeShoulderSuitcase_1 : Subsystem  Tag=actuator/ColorRegion  Priority=0  LoadFcn=load('PrescanColorData')  mask(PreScan Sink Block: VisuTextureColor){}
      mask help: The VisuTextureColor block provides a way to adapt the color of a vehicle. For more information, please click Help.
      settings: OpenFcn=open_system([gcb '/Actuator'],'mask')
      mask Help: eval('openHelp(230)')
      mask Display: image(imread('TextureColor.png'))
  VISUColorRegion_Lower_Body_Male_Old_White_WithStick_1 : Subsystem  Tag=actuator/ColorRegion  Priority=0  LoadFcn=load('PrescanColorData')  mask(PreScan Sink Block: VisuTextureColor){}
      mask help: The VisuTextureColor block provides a way to adapt the color of a vehicle. For more information, please click Help.
      settings: OpenFcn=open_system([gcb '/Actuator'],'mask')
      mask Help: eval('openHelp(230)')
      mask Display: image(imread('TextureColor.png'))
  VISUColorRegion_Lower_Body_Male_Old_White_WithWalkerWithWheels_1 : Subsystem  Tag=actuator/ColorRegion  Priority=0  LoadFcn=load('PrescanColorData')  mask(PreScan Sink Block: VisuTextureColor){}
      mask help: The VisuTextureColor block provides a way to adapt the color of a vehicle. For more information, please click Help.
      settings: OpenFcn=open_system([gcb '/Actuator'],'mask')
      mask Help: eval('openHelp(230)')
      mask Display: image(imread('TextureColor.png'))
  VISUColorRegion_Lower_Body_Male_Overweight_1 : Subsystem  Tag=actuator/ColorRegion  Priority=0  LoadFcn=load('PrescanColorData')  mask(PreScan Sink Block: VisuTextureColor){}
      mask help: The VisuTextureColor block provides a way to adapt the color of a vehicle. For more information, please click Help.
      settings: OpenFcn=open_system([gcb '/Actuator'],'mask')
      mask Help: eval('openHelp(230)')
      mask Display: image(imread('TextureColor.png'))
  VISUColorRegion_Lower_Body_Male_ShoppingBag_1 : Subsystem  Tag=actuator/ColorRegion  Priority=0  LoadFcn=load('PrescanColorData')  mask(PreScan Sink Block: VisuTextureColor){}
      mask help: The VisuTextureColor block provides a way to adapt the color of a vehicle. For more information, please click Help.
      settings: OpenFcn=open_system([gcb '/Actuator'],'mask')
      mask Help: eval('openHelp(230)')
      mask Display: image(imread('TextureColor.png'))
  VISUColorRegion_Lower_Body_Male_wBackpack_1 : Subsystem  Tag=actuator/ColorRegion  Priority=0  LoadFcn=load('PrescanColorData')  mask(PreScan Sink Block: VisuTextureColor){}
      mask help: The VisuTextureColor block provides a way to adapt the color of a vehicle. For more information, please click Help.
      settings: OpenFcn=open_system([gcb '/Actuator'],'mask')
      mask Help: eval('openHelp(230)')
      mask Display: image(imread('TextureColor.png'))
  VISUColorRegion_Lower_Body_Male_wLargeBackpack_1 : Subsystem  Tag=actuator/ColorRegion  Priority=0  LoadFcn=load('PrescanColorData')  mask(PreScan Sink Block: VisuTextureColor){}
      mask help: The VisuTextureColor block provides a way to adapt the color of a vehicle. For more information, please click Help.
